simulink model "CONTROL_01"  (R2018b)
settings: Solver=FixedStepAuto  StartTime=0.0  StopTime=30  FixedStep=0.01  RelTol=1e-3
model workspace: external: MATLAB File D:\OneDrive\STUDY\RIC LAB\PROJECT 6DOF\CODE\CODE 6DOF\07_CONTROL\CONTROL_02\ROBOT_DataFile.m (data not in the file)
undefined symbols (not defined in the file or in its folder): smiData, X, Y, Z
libraries: sm_lib x35, nesl_utility x7
(part 76 of 185)

== matlab function CONTROL_01/6DOF Manipulator4/Dynamics ==
  data: t input; Fe input; dthe input; the input; Fv input; Fc input; ddthe output; m input; L input; Pic input; dt output; ex output; I input
function [ddthe,dt,ex] = DYN_6DOF(t,Fe,dthe,the,Fv,Fc,m,L,Pic,I)
e1 = the(1); e2 = the(2); e3 = the(3);
e4 = the(4); e5 = the(5); e6 = the(6);
de1 = dthe(1); de2 = dthe(2); de3 = dthe(3);
de4 = dthe(4); de5 = dthe(5); de6 = dthe(6);
x1 = Pic(1,1); y1 = Pic(1,2); z1 = Pic(1,3);
x2 = Pic(2,1); y2 = Pic(2,2); z2 = Pic(2,3);
x3 = Pic(3,1); y3 = Pic(3,2); z3 = Pic(3,3);
x4 = Pic(4,1); y4 = Pic(4,2); z4 = Pic(4,3);
x5 = Pic(5,1); y5 = Pic(5,2); z5 = Pic(5,3);
x6 = Pic(6,1); y6 = Pic(6,2); z6 = Pic(6,3);
I1xx = I(1,1); I1yy = I(1,2); I1zz = I(1,3);
I1xy = I(1,4); I1yz = I(1,5); I1zx = I(1,6);
I2xx = I(2,1); I2yy = I(2,2); I2zz = I(2,3);
I2xy = I(2,4); I2yz = I(2,5); I2zx = I(2,6);
I3xx = I(3,1); I3yy = I(3,2); I3zz = I(3,3);
I3xy = I(3,4); I3yz = I(3,5); I3zx = I(3,6);
I4xx = I(4,1); I4yy = I(4,2); I4zz = I(4,3);
I4xy = I(4,4); I4yz = I(4,5); I4zx = I(4,6);
I5xx = I(5,1); I5yy = I(5,2); I5zz = I(5,3);
I5xy = I(5,4); I5yz = I(5,5); I5zx = I(5,6);
I6xx = I(6,1); I6yy = I(6,2); I6zz = I(6,3);
I6xy = I(6,4); I6yz = I(6,5); I6zx = I(6,6);
a1 = L(1); a2 = L(2); a3 = L(3); d1 = L(4); d4 = L(5); d7 = L(6);
m1 = m(1); m2 = m(2); m3 = m(3); m4 = m(4); m5 = m(5); m6 = m(6);
g = -9.80665;
%% 
M = ...
[I1zz + m3*(cos(e1)*(a1 + a2*sin(e2)) - z3*sin(e1) + y3*cos(e2 + e3)*cos(e1) + x3*sin(e2 + e3)*cos(e1))^2 + m6*(sin(e1)*(a1 + d4*cos(e2 + e3) + a3*sin(e2 + e3) + a2*sin(e2)) - x6*(sin(e6)*(cos(e1)*cos(e4) + sin(e2 + e3)*sin(e1)*sin(e4)) + cos(e6)*(cos(e5)*(cos(e1)*sin(e4) - sin(e2 + e3)*cos(e4)*sin(e1)) - cos(e2 + e3)*sin(e1)*sin(e5))) - y6*(cos(e6)*(cos(e1)*cos(e4) + sin(e2 + e3)*sin(e1)*sin(e4)) - sin(e6)*(cos(e5)*(cos(e1)*sin(e4) - sin(e2 + e3)*cos(e4)*sin(e1)) - cos(e2 + e3)*sin(e1)*sin(e5))) + z6*(sin(e5)*(cos(e1)*sin(e4) - sin(e2 + e3)*cos(e4)*sin(e1)) + cos(e2 + e3)*cos(e5)*sin(e1)))^2 + (I6xx*(cos(e2)*cos(e3)*sin(e4)*sin(e6) + cos(e2)*cos(e6)*sin(e3)*sin(e5) + cos(e3)*cos(e6)*sin(e2)*sin(e5) - sin(e2)*sin(e3)*sin(e4)*sin(e6) - cos(e2)*cos(e3)*cos(e4)*cos(e5)*cos(e6) + cos(e4)*cos(e5)*cos(e6)*sin(e2)*sin(e3)) + I6xy*(cos(e6)*sin(e2)*sin(e3)*sin(e4) - cos(e2)*cos(e3)*cos(e6)*sin(e4) + cos(e2)*sin(e3)*sin(e5)*sin(e6) + cos(e3)*sin(e2)*sin(e5)*sin(e6) - cos(e2)*cos(e3)*cos(e4)*cos(e5)*sin(e6) + cos(e4)*cos(e5)*sin(e2)*sin(e3)*sin(e6)) - I6zx*(cos(e2)*cos(e5)*sin(e3) + cos(e3)*cos(e5)*sin(e2) + cos(e2)*cos(e3)*cos(e4)*sin(e5) - cos(e4)*sin(e2)*sin(e3)*sin(e5)))*(cos(e2)*cos(e3)*sin(e4)*sin(e6) + cos(e2)*cos(e6)*sin(e3)*sin(e5) + cos(e3)*cos(e6)*sin(e2)*sin(e5) - sin(e2)*sin(e3)*sin(e4)*sin(e6) - cos(e2)*cos(e3)*cos(e4)*cos(e5)*cos(e6) + cos(e4)*cos(e5)*cos(e6)*sin(e2)*sin(e3)) + (cos(e2)*cos(e3)*sin(e4) - sin(e2)*sin(e3)*sin(e4))*(I5zz*(cos(e2)*cos(e3)*sin(e4) - sin(e2)*sin(e3)*sin(e4)) + I5yz*(cos(e2)*cos(e5)*sin(e3) + cos(e3)*cos(e5)*sin(e2) + cos(e2)*cos(e3)*cos(e4)*sin(e5) - cos(e4)*sin(e2)*sin(e3)*sin(e5)) + I5zx*(cos(e2)*sin(e3)*sin(e5) + cos(e3)*sin(e2)*sin(e5) - cos(e2)*cos(e3)*cos(e4)*cos(e5) + cos(e4)*cos(e5)*sin(e2)*sin(e3))) + (cos(e2)*cos(e3)*cos(e4) - cos(e4)*sin(e2)*sin(e3))*(I4zx*sin(e2 + e3) + I4xx*(cos(e2)*cos(e3)*cos(e4) - cos(e4)*sin(e2)*sin(e3)) + I4xy*(cos(e2)*cos(e3)*sin(e4) - sin(e2)*sin(e3)*sin(e4))) + m3*(sin(e1)*(a1 + a2*sin(e2)) + z3*cos(e1) + y3*cos(e2 + e3)*sin(e1) + x3*sin(e2 + e3)*sin(e1))^2 + (I6xy*(cos(e2)*cos(e3)*sin(e4)*sin(e6) + cos(e2)*cos(e6)*sin(e3)*sin(e5) + cos(e3)*cos(e6)*sin(e2)*sin(e5) - sin(e2)*sin(e3)*sin(e4)*sin(e6) - cos(e2)*cos(e3)*cos(e4)*cos(e5)*cos(e6) + cos(e4)*cos(e5)*cos(e6)*sin(e2)*sin(e3)) + I6yy*(cos(e6)*sin(e2)*sin(e3)*sin(e4) - cos(e2)*cos(e3)*cos(e6)*sin(e4) + cos(e2)*sin(e3)*sin(e5)*sin(e6) + cos(e3)*sin(e2)*sin(e5)*sin(e6) - cos(e2)*cos(e3)*cos(e4)*cos(e5)*sin(e6) + cos(e4)*cos(e5)*sin(e2)*sin(e3)*sin(e6)) + I6yz*(cos(e2)*cos(e5)*sin(e3) + cos(e3)*cos(e5)*sin(e2) + cos(e2)*cos(e3)*cos(e4)*sin(e5) - cos(e4)*sin(e2)*sin(e3)*sin(e5)))*(cos(e6)*sin(e2)*sin(e3)*sin(e4) - cos(e2)*cos(e3)*cos(e6)*sin(e4) + cos(e2)*sin(e3)*sin(e5)*sin(e6) + cos(e3)*sin(e2)*sin(e5)*sin(e6) - cos(e2)*cos(e3)*cos(e4)*cos(e5)*sin(e6) + cos(e4)*cos(e5)*sin(e2)*sin(e3)*sin(e6)) + (I5zx*(cos(e2)*cos(e3)*sin(e4) - sin(e2)*sin(e3)*sin(e4)) + I5xx*(cos(e2)*sin(e3)*sin(e5) + cos(e3)*sin(e2)*sin(e5) - cos(e2)*cos(e3)*cos(e4)*cos(e5) + cos(e4)*cos(e5)*sin(e2)*sin(e3)) - I5xy*(cos(e2)*cos(e5)*sin(e3) + cos(e3)*cos(e5)*sin(e2) + cos(e2)*cos(e3)*cos(e4)*sin(e5) - cos(e4)*sin(e2)*sin(e3)*sin(e5)))*(cos(e2)*sin(e3)*sin(e5) + cos(e3)*sin(e2)*sin(e5) - cos(e2)*cos(e3)*cos(e4)*cos(e5) + cos(e4)*cos(e5)*sin(e2)*sin(e3)) + (I5yz*(cos(e2)*cos(e3)*sin(e4) - sin(e2)*sin(e3)*sin(e4)) - I5xy*(cos(e2)*sin(e3)*sin(e5) + cos(e3)*sin(e2)*sin(e5) - cos(e2)*cos(e3)*cos(e4)*cos(e5) + cos(e4)*cos(e5)*sin(e2)*sin(e3)) + I5yy*(cos(e2)*cos(e5)*sin(e3) + cos(e3)*cos(e5)*sin(e2) + cos(e2)*cos(e3)*cos(e4)*sin(e5) - cos(e4)*sin(e2)*sin(e3)*sin(e5)))*(cos(e2)*cos(e5)*sin(e3) + cos(e3)*cos(e5)*sin(e2) + cos(e2)*cos(e3)*cos(e4)*sin(e5) - cos(e4)*sin(e2)*sin(e3)*sin(e5)) + m5*(cos(e1)*(a1 + d4*cos(e2 + e3) + a3*sin(e2 + e3) + a2*sin(e2)) - z5*(cos(e4)*sin(e1) - sin(e2 + e3)*cos(e1)*sin(e4)) + x5*(cos(e5)*(sin(e1)*sin(e4) + sin(e2 + e3)*cos(e1)*cos(e4)) + cos(e2 + e3)*cos(e1)*sin(e5)) - y5*(sin(e5)*(sin(e1)*sin(e4) + sin(e2 + e3)*cos(e1)*cos(e4)) - cos(e2 + e3)*cos(e1)*cos(e5)))^2 + (cos(e2)*cos(e3)*sin(e4) - sin(e2)*sin(e3)*sin(e4))*(I4xy*(cos(e2)*cos(e3)*cos(e4) - cos(e4)*sin(e2)*sin(e3)) - I4yz*sin(e2 + e3) + I4yy*(cos(e2)*cos(e3)*sin(e4) - sin(e2)*sin(e3)*sin(e4))) + cos(e2)*(I2xx*cos(e2) + I2xy*sin(e2)) + sin(e2)*(I2xy*cos(e2) + I2yy*sin(e2)) + m4*(cos(e1)*(a1 + d4*cos(e2 + e3) + a3*sin(e2 + e3) + a2*sin(e2)) + x4*(sin(e1)*sin(e4) + sin(e2 + e3)*cos(e1)*cos(e4)) + y4*(cos(e4)*sin(e1) - sin(e2 + e3)*cos(e1)*sin(e4)) + z4*cos(e2 + e3)*cos(e1))^2 + m5*(sin(e1)*(a1 + d4*cos(e2 + e3) + a3*sin(e2 + e3) + a2*sin(e2)) + z5*(cos(e1)*cos(e4) + sin(e2 + e3)*sin(e1)*sin(e4)) - x5*(cos(e5)*(cos(e1)*sin(e4) - sin(e2 + e3)*cos(e4)*sin(e1)) - cos(e2 + e3)*sin(e1)*sin(e5)) + y5*(sin(e5)*(cos(e1)*sin(e4) - sin(e2 + e3)*cos(e4)*sin(e1)) + cos(e2 + e3)*cos(e5)*sin(e1)))^2 + m2*(a1*cos(e1) - z2*sin(e1) + y2*cos(e1)*cos(e2) + x2*cos(e1)*sin(e2))^2 + (I6yz*(cos(e6)*sin(e2)*sin(e3)*sin(e4) - cos(e2)*cos(e3)*cos(e6)*sin(e4) + cos(e2)*sin(e3)*sin(e5)*sin(e6) + cos(e3)*sin(e2)*sin(e5)*sin(e6) - cos(e2)*cos(e3)*cos(e4)*cos(e5)*sin(e6) + cos(e4)*cos(e5)*sin(e2)*sin(e3)*sin(e6)) - I6zx*(cos(e2)*cos(e3)*sin(e4)*sin(e6) + cos(e2)*cos(e6)*sin(e3)*sin(e5) + cos(e3)*cos(e6)*sin(e2)*sin(e5) - sin(e2)*sin(e3)*sin(e4)*sin(e6) - cos(e2)*cos(e3)*cos(e4)*cos(e5)*cos(e6) + cos(e4)*cos(e5)*cos(e6)*sin(e2)*sin(e3)) + I6zz*(cos(e2)*cos(e5)*sin(e3) + cos(e3)*cos(e5)*sin(e2) + cos(e2)*cos(e3)*cos(e4)*sin(e5) - cos(e4)*sin(e2)*sin(e3)*sin(e5)))*(cos(e2)*cos(e5)*sin(e3) + cos(e3)*cos(e5)*sin(e2) + cos(e2)*cos(e3)*cos(e4)*sin(e5) - cos(e4)*sin(e2)*sin(e3)*sin(e5)) + m4*(sin(e1)*(a1 + d4*cos(e2 + e3) + a3*sin(e2 + e3) + a2*sin(e2)) - x4*(cos(e1)*sin(e4) - sin(e2 + e3)*cos(e4)*sin(e1)) - y4*(cos(e1)*cos(e4) + sin(e2 + e3)*sin(e1)*sin(e4)) + z4*cos(e2 + e3)*sin(e1))^2 + cos(e2 + e3)*(I3xx*cos(e2 + e3) + I3xy*sin(e2 + e3)) + m2*(a1*sin(e1) + z2*cos(e1) + y2*cos(e2)*sin(e1) + x2*sin(e1)*sin(e2))^2 + sin(e2 + e3)*(I3xy*cos(e2 + e3) + I3yy*sin(e2 + e3)) + m1*(y1*cos(e1) + x1*sin(e1))^2 + m1*(x1*cos(e1) - y1*sin(e1))^2 + m6*(cos(e1)*(a1 + d4*cos(e2 + e3) + a3*sin(e2 + e3) + a2*sin(e2)) + x6*(sin(e6)*(cos(e4)*sin(e1) - sin(e2 + e3)*cos(e1)*sin(e4)) + cos(e6)*(cos(e5)*(sin(e1)*sin(e4) + sin(e2 + e3)*cos(e1)*cos(e4)) + cos(e2 + e3)*cos(e1)*sin(e5))) + y6*(cos(e6)*(cos(e4)*sin(e1) - sin(e2 + e3)*cos(e1)*sin(e4)) - sin(e6)*(cos(e5)*(sin(e1)*sin(e4) + sin(e2 + e3)*cos(e1)*cos(e4)) + cos(e2 + e3)*cos(e1)*sin(e5))) - z6*(sin(e5)*(sin(e1)*sin(e4) + sin(e2 + e3)*cos(e1)*cos(e4)) - cos(e2 + e3)*cos(e1)*cos(e5)))^2 + sin(e2 + e3)*(I4zz*sin(e2 + e3) + I4zx*(cos(e2)*cos(e3)*cos(e4) - cos(e4)*sin(e2)*sin(e3)) - I4yz*(cos(e2)*cos(e3)*sin(e4) - sin(e2)*sin(e3)*sin(e4))),cos(e4)*(I4xy*(cos(e2)*cos(e3)*cos(e4) - cos(e4)*sin(e2)*sin(e3)) - I4yz*sin(e2 + e3) + I4yy*(cos(e2)*cos(e3)*sin(e4) - sin(e2)*sin(e3)*sin(e4))) - sin(e4)*(I4zx*sin(e2 + e3) + I4xx*(cos(e2)*cos(e3)*cos(e4) - cos(e4)*sin(e2)*sin(e3)) + I4xy*(cos(e2)*cos(e3)*sin(e4) - sin(e2)*sin(e3)*sin(e4))) - I3zx*cos(e2 + e3) + I3yz*sin(e2 + e3) - I2zx*cos(e2) + I2yz*sin(e2) + (cos(e4)*sin(e6) + cos(e5)*cos(e6)*sin(e4))*(I6xx*(cos(e2)*cos(e3)*sin(e4)*sin(e6) + cos(e2)*cos(e6)*sin(e3)*sin(e5) + cos(e3)*cos(e6)*sin(e2)*sin(e5) - sin(e2)*sin(e3)*sin(e4)*sin(e6) - cos(e2)*cos(e3)*cos(e4)*cos(e5)*cos(e6) + cos(e4)*cos(e5)*cos(e6)*sin(e2)*sin(e3)) + I6xy*(cos(e6)*sin(e2)*sin(e3)*sin(e4) - cos(e2)*cos(e3)*cos(e6)*sin(e4) + cos(e2)*sin(e3)*sin(e5)*sin(e6) + cos(e3)*sin(e2)*sin(e5)*sin(e6) - cos(e2)*cos(e3)*cos(e4)*cos(e5)*sin(e6) + cos(e4)*cos(e5)*sin(e2)*sin(e3)*sin(e6)) - I6zx*(cos(e2)*cos(e5)*sin(e3) + cos(e3)*cos(e5)*sin(e2) + cos(e2)*cos(e3)*cos(e4)*sin(e5) - cos(e4)*sin(e2)*sin(e3)*sin(e5))) - (cos(e4)*cos(e6) - cos(e5)*sin(e4)*sin(e6))*(I6xy*(cos(e2)*cos(e3)*sin(e4)*sin(e6) + cos(e2)*cos(e6)*sin(e3)*sin(e5) + cos(e3)*cos(e6)*sin(e2)*sin(e5) - sin(e2)*sin(e3)*sin(e4)*sin(e6) - cos(e2)*cos(e3)*cos(e4)*cos(e5)*cos(e6) + cos(e4)*cos(e5)*cos(e6)*sin(e2)*sin(e3)) + I6yy*(cos(e6)*sin(e2)*sin(e3)*sin(e4) - cos(e2)*cos(e3)*cos(e6)*sin(e4) + cos(e2)*sin(e3)*sin(e5)*sin(e6) + cos(e3)*sin(e2)*sin(e5)*sin(e6) - cos(e2)*cos(e3)*cos(e4)*cos(e5)*sin(e6) + cos(e4)*cos(e5)*sin(e2)*sin(e3)*sin(e6)) + I6yz*(cos(e2)*cos(e5)*sin(e3) + cos(e3)*cos(e5)*sin(e2) + cos(e2)*cos(e3)*cos(e4)*sin(e5) - cos(e4)*sin(e2)*sin(e3)*sin(e5))) + cos(e4)*(I5zz*(cos(e2)*cos(e3)*sin(e4) - sin(e2)*sin(e3)*sin(e4)) + I5yz*(cos(e2)*cos(e5)*sin(e3) + cos(e3)*cos(e5)*sin(e2) + cos(e2)*cos(e3)*cos(e4)*sin(e5) - cos(e4)*sin(e2)*sin(e3)*sin(e5)) + I5zx*(cos(e2)*sin(e3)*sin(e5) + cos(e3)*sin(e2)*sin(e5) - cos(e2)*cos(e3)*cos(e4)*cos(e5) + cos(e4)*cos(e5)*sin(e2)*sin(e3))) - m3*(x3*cos(e2 + e3)*cos(e1) - y3*sin(e2 + e3)*cos(e1) + a2*cos(e1)*cos(e2))*(sin(e1)*(a1 + a2*sin(e2)) + z3*cos(e1) + y3*cos(e2 + e3)*sin(e1) + x3*sin(e2 + e3)*sin(e1)) + m3*(x3*cos(e2 + e3)*sin(e1) - y3*sin(e2 + e3)*sin(e1) + a2*cos(e2)*sin(e1))*(cos(e1)*(a1 + a2*sin(e2)) - z3*sin(e1) + y3*cos(e2 + e3)*cos(e1) + x3*sin(e2 + e3)*cos(e1)) + m6*(sin(e1)*(a1 + d4*cos(e2 + e3) + a3*sin(e2 + e3) + a2*sin(e2)) - x6*(sin(e6)*(cos(e1)*cos(e4) + sin(e2 + e3)*sin(e1)*sin(e4)) + cos(e6)*(cos(e5)*(cos(e1)*sin(e4) - sin(e2 + e3)*cos(e4)*sin(e1)) - cos(e2 + e3)*sin(e1)*sin(e5))) - y6*(cos(e6)*(cos(e1)*cos(e4) + sin(e2 + e3)*sin(e1)*sin(e4)) - sin(e6)*(cos(e5)*(cos(e1)*sin(e4) - sin(e2 + e3)*cos(e4)*sin(e1)) - cos(e2 + e3)*sin(e1)*sin(e5))) + z6*(sin(e5)*(cos(e1)*sin(e4) - sin(e2 + e3)*cos(e4)*sin(e1)) + cos(e2 + e3)*cos(e5)*sin(e1)))*(x6*(cos(e6)*(sin(e2 + e3)*cos(e1)*sin(e5) - cos(e2 + e3)*cos(e1)*cos(e4)*cos(e5)) + cos(e2 + e3)*cos(e1)*sin(e4)*sin(e6)) - y6*(sin(e6)*(sin(e2 + e3)*cos(e1)*sin(e5) - cos(e2 + e3)*cos(e1)*cos(e4)*cos(e5)) - cos(e2 + e3)*cos(e1)*cos(e6)*sin(e4)) + z6*(sin(e2 + e3)*cos(e1)*cos(e5) + cos(e2 + e3)*cos(e1)*cos(e4)*sin(e5)) - cos(e1)*(a3*cos(e2 + e3) - d4*sin(e2 + e3) + a2*cos(e2))) - sin(e4)*sin(e5)*(I6yz*(cos(e6)*sin(e2)*sin(e3)*sin(e4) - cos(e2)*cos(e3)*cos(e6)*sin(e4) + cos(e2)*sin(e3)*sin(e5)*sin(e6) + cos(e3)*sin(e2)*sin(e5)*sin(e6) - cos(e2)*cos(e3)*cos(e4)*cos(e5)*sin(e6) + cos(e4)*cos(e5)*sin(e2)*sin(e3)*sin(e6)) - I6zx*(cos(e2)*cos(e3)*sin(e4)*sin(e6) + cos(e2)*cos(e6)*sin(e3)*sin(e5) + cos(e3)*cos(e6)*sin(e2)*sin(e5) - sin(e2)*sin(e3)*sin(e4)*sin(e6) - cos(e2)*cos(e3)*cos(e4)*cos(e5)*cos(e6) + cos(e4)*cos(e5)*cos(e6)*sin(e2)*sin(e3)) + I6zz*(cos(e2)*cos(e5)*sin(e3) + cos(e3)*cos(e5)*sin(e2) + cos(e2)*cos(e3)*cos(e4)*sin(e5) - cos(e4)*sin(e2)*sin(e3)*sin(e5))) - m6*(cos(e1)*(a1 + d4*cos(e2 + e3) + a3*sin(e2 + e3) + a2*sin(e2)) + x6*(sin(e6)*(cos(e4)*sin(e1) - sin(e2 + e3)*cos(e1)*sin(e4)) + cos(e6)*(cos(e5)*(sin(e1)*sin(e4) + sin(e2 + e3)*cos(e1)*cos(e4)) + cos(e2 + e3)*cos(e1)*sin(e5))) + y6*(cos(e6)*(cos(e4)*sin(e1) - sin(e2 + e3)*cos(e1)*sin(e4)) - sin(e6)*(cos(e5)*(sin(e1)*sin(e4) + sin(e2 + e3)*cos(e1)*cos(e4)) + cos(e2 + e3)*cos(e1)*sin(e5))) - z6*(sin(e5)*(sin(e1)*sin(e4) + sin(e2 + e3)*cos(e1)*cos(e4)) - cos(e2 + e3)*cos(e1)*cos(e5)))*(x6*(cos(e6)*(sin(e2 + e3)*sin(e1)*sin(e5) - cos(e2 + e3)*cos(e4)*cos(e5)*sin(e1)) + cos(e2 + e3)*sin(e1)*sin(e4)*sin(e6)) - y6*(sin(e6)*(sin(e2 + e3)*sin(e1)*sin(e5) - cos(e2 + e3)*cos(e4)*cos(e5)*sin(e1)) - cos(e2 + e3)*cos(e6)*sin(e1)*sin(e4)) + z6*(sin(e2 + e3)*cos(e5)*sin(e1) + cos(e2 + e3)*cos(e4)*sin(e1)*sin(e5)) - sin(e1)*(a3*cos(e2 + e3) - d4*sin(e2 + e3) + a2*cos(e2))) + m5*(x5*(sin(e2 + e3)*cos(e1)*sin(e5) - cos(e2 + e3)*cos(e1)*cos(e4)*cos(e5)) + y5*(sin(e2 + e3)*cos(e1)*cos(e5) + cos(e2 + e3)*cos(e1)*cos(e4)*sin(e5)) - cos(e1)*(a3*cos(e2 + e3) - d4*sin(e2 + e3) + a2*cos(e2)) - z5*cos(e2 + e3)*cos(e1)*sin(e4))*(sin(e1)*(a1 + d4*cos(e2 + e3) + a3*sin(e2 + e3) + a2*sin(e2)) + z5*(cos(e1)*cos(e4) + sin(e2 + e3)*sin(e1)*sin(e4)) - x5*(cos(e5)*(cos(e1)*sin(e4) - sin(e2 + e3)*cos(e4)*sin(e1)) - cos(e2 + e3)*sin(e1)*sin(e5)) + y5*(sin(e5)*(cos(e1)*sin(e4) - sin(e2 + e3)*cos(e4)*sin(e1)) + cos(e2 + e3)*cos(e5)*sin(e1))) - m2*(x2*cos(e1)*cos(e2) - y2*cos(e1)*sin(e2))*(a1*sin(e1) + z2*cos(e1) + y2*cos(e2)*sin(e1) + x2*sin(e1)*sin(e2)) + m2*(x2*cos(e2)*sin(e1) - y2*sin(e1)*sin(e2))*(a1*cos(e1) - z2*sin(e1) + y2*cos(e1)*cos(e2) + x2*cos(e1)*sin(e2)) - m4*(cos(e1)*(a3*cos(e2 + e3) - d4*sin(e2 + e3) + a2*cos(e2)) - z4*sin(e2 + e3)*cos(e1) - y4*cos(e2 + e3)*cos(e1)*sin(e4) + x4*cos(e2 + e3)*cos(e1)*cos(e4))*(sin(e1)*(a1 + d4*cos(e2 + e3) + a3*sin(e2 + e3) + a2*sin(e2)) - x4*(cos(e1)*sin(e4) - sin(e2 + e3)*cos(e4)*sin(e1)) - y4*(cos(e1)*cos(e4) + sin(e2 + e3)*sin(e1)*sin(e4)) + z4*cos(e2 + e3)*sin(e1)) - m5*(cos(e1)*(a1 + d4*cos(e2 + e3) + a3*sin(e2 + e3) + a2*sin(e2)) - z5*(cos(e4)*sin(e1) - sin(e2 + e3)*cos(e1)*sin(e4)) + x5*(cos(e5)*(sin(e1)*sin(e4) + sin(e2 + e3)*cos(e1)*cos(e4)) + cos(e2 + e3)*cos(e1)*sin(e5)) - y5*(sin(e5)*(sin(e1)*sin(e4) + sin(e2 + e3)*cos(e1)*cos(e4)) - cos(e2 + e3)*cos(e1)*cos(e5)))*(x5*(sin(e2 + e3)*sin(e1)*sin(e5) - cos(e2 + e3)*cos(e4)*cos(e5)*sin(e1)) + y5*(sin(e2 + e3)*cos(e5)*sin(e1) + cos(e2 + e3)*cos(e4)*sin(e1)*sin(e5)) - sin(e1)*(a3*cos(e2 + e3) - d4*sin(e2 + e3) + a2*cos(e2)) - z5*cos(e2 + e3)*sin(e1)*sin(e4)) + m4*(cos(e1)*(a1 + d4*cos(e2 + e3) + a3*sin(e2 + e3) + a2*sin(e2)) + x4*(sin(e1)*sin(e4) + sin(e2 + e3)*cos(e1)*cos(e4)) + y4*(cos(e4)*sin(e1) - sin(e2 + e3)*cos(e1)*sin(e4)) + z4*cos(e2 + e3)*cos(e1))*(sin(e1)*(a3*cos(e2 + e3) - d4*sin(e2 + e3) + a2*cos(e2)) - z4*sin(e2 + e3)*sin(e1) + x4*cos(e2 + e3)*cos(e4)*sin(e1) - y4*cos(e2 + e3)*sin(e1)*sin(e4)) + cos(e5)*sin(e4)*(I5zx*(cos(e2)*cos(e3)*sin(e4) - sin(e2)*sin(e3)*sin(e4)) + I5xx*(cos(e2)*sin(e3)*sin(e5) + cos(e3)*sin(e2)*sin(e5) - cos(e2)*cos(e3)*cos(e4)*cos(e5) + cos(e4)*cos(e5)*sin(e2)*sin(e3)) - I5xy*(cos(e2)*cos(e5)*sin(e3) + cos(e3)*cos(e5)*sin(e2) + cos(e2)*cos(e3)*cos(e4)*sin(e5) - cos(e4)*sin(e2)*sin(e3)*sin(e5))) - sin(e4)*sin(e5)*(I5yz*(cos(e2)*cos(e3)*sin(e4) - sin(e2)*sin(e3)*sin(e4)) - I5xy*(cos(e2)*sin(e3)*sin(e5) + cos(e3)*sin(e2)*sin(e5) - cos(e2)*cos(e3)*cos(e4)*cos(e5) + cos(e4)*cos(e5)*sin(e2)*sin(e3)) + I5yy*(cos(e2)*cos(e5)*sin(e3) + cos(e3)*cos(e5)*sin(e2) + cos(e2)*cos(e3)*cos(e4)*sin(e5) - cos(e4)*sin(e2)*sin(e3)*sin(e5))),cos(e4)*(I4xy*(cos(e2)*cos(e3)*cos(e4) - cos(e4)*sin(e2)*sin(e3)) - I4yz*sin(e2 + e3) + I4yy*(cos(e2)*cos(e3)*sin(e4) - sin(e2)*sin(e3)*sin(e4))) - sin(e4)*(I4zx*sin(e2 + e3) + I4xx*(cos(e2)*cos(e3)*cos(e4) - cos(e4)*sin(e2)*sin(e3)) + I4xy*(cos(e2)*cos(e3)*sin(e4) - sin(e2)*sin(e3)*sin(e4))) - I3zx*cos(e2 + e3) + I3yz*sin(e2 + e3) + (cos(e4)*sin(e6) + cos(e5)*cos(e6)*sin(e4))*(I6xx*(cos(e2)*cos(e3)*sin(e4)*sin(e6) + cos(e2)*cos(e6)*sin(e3)*sin(e5) + cos(e3)*cos(e6)*sin(e2)*sin(e5) - sin(e2)*sin(e3)*sin(e4)*sin(e6) - cos(e2)*cos(e3)*cos(e4)*cos(e5)*cos(e6) + cos(e4)*cos(e5)*cos(e6)*sin(e2)*sin(e3)) + I6xy*(cos(e6)*sin(e2)*sin(e3)*sin(e4) - cos(e2)*cos(e3)*cos(e6)*sin(e4) + cos(e2)*sin(e3)*sin(e5)*sin(e6) + cos(e3)*sin(e2)*sin(e5)*sin(e6) - cos(e2)*cos(e3)*cos(e4)*cos(e5)*sin(e6) + cos(e4)*cos(e5)*sin(e2)*sin(e3)*sin(e6)) - I6zx*(cos(e2)*cos(e5)*sin(e3) + cos(e3)*cos(e5)*sin(e2) + cos(e2)*cos(e3)*cos(e4)*sin(e5) - cos(e4)*sin(e2)*sin(e3)*sin(e5))) - (cos(e4)*cos(e6) - cos(e5)*sin(e4)*sin(e6))*(I6xy*(cos(e2)*cos(e3)*sin(e4)*sin(e6) + cos(e2)*cos(e6)*sin(e3)*sin(e5) + cos(e3)*cos(e6)*sin(e2)*sin(e5) - sin(e2)*sin(e3)*sin(e4)*sin(e6) - cos(e2)*cos(e3)*cos(e4)*cos(e5)*cos(e6) + cos(e4)*cos(e5)*cos(e6)*sin(e2)*sin(e3)) + I6yy*(cos(e6)*sin(e2)*sin(e3)*sin(e4) - cos(e2)*cos(e3)*cos(e6)*sin(e4) + cos(e2)*sin(e3)*sin(e5)*sin(e6) + cos(e3)*sin(e2)*sin(e5)*sin(e6) - cos(e2)*cos(e3)*cos(e4)*cos(e5)*sin(e6) + cos(e4)*cos(e5)*sin(e2)*sin(e3)*sin(e6)) + I6yz*(cos(e2)*cos(e5)*sin(e3) + cos(e3)*cos(e5)*sin(e2) + cos(e2)*cos(e3)*cos(e4)*sin(e5) - cos(e4)*sin(e2)*sin(e3)*sin(e5))) + cos(e4)*(I5zz*(cos(e2)*cos(e3)*sin(e4) - sin(e2)*sin(e3)*sin(e4)) + I5yz*(cos(e2)*cos(e5)*sin(e3) + cos(e3)*cos(e5)*sin(e2) + cos(e2)*cos(e3)*cos(e4)*sin(e5) - cos(e4)*sin(e2)*sin(e3)*sin(e5)) + I5zx*(cos(e2)*sin(e3)*sin(e5) + cos(e3)*sin(e2)*sin(e5) - cos(e2)*cos(e3)*cos(e4)*cos(e5) + cos(e4)*cos(e5)*sin(e2)*sin(e3))) + m5*(sin(e1)*(a1 + d4*cos(e2 + e3) + a3*sin(e2 + e3) + a2*sin(e2)) + z5*(cos(e1)*cos(e4) + sin(e2 + e3)*sin(e1)*sin(e4)) - x5*(cos(e5)*(cos(e1)*sin(e4) - sin(e2 + e3)*cos(e4)*sin(e1)) - cos(e2 + e3)*sin(e1)*sin(e5)) + y5*(sin(e5)*(cos(e1)*sin(e4) - sin(e2 + e3)*cos(e4)*sin(e1)) + cos(e2 + e3)*cos(e5)*sin(e1)))*(x5*(sin(e2 + e3)*cos(e1)*sin(e5) - cos(e2 + e3)*cos(e1)*cos(e4)*cos(e5)) + y5*(sin(e2 + e3)*cos(e1)*cos(e5) + cos(e2 + e3)*cos(e1)*cos(e4)*sin(e5)) - cos(e1)*(a3*cos(e2 + e3) - d4*sin(e2 + e3)) - z5*cos(e2 + e3)*cos(e1)*sin(e4)) - m4*(sin(e1)*(a1 + d4*cos(e2 + e3) + a3*sin(e2 + e3) + a2*sin(e2)) - x4*(cos(e1)*sin(e4) - sin(e2 + e3)*cos(e4)*sin(e1)) - y4*(cos(e1)*cos(e4) + sin(e2 + e3)*sin(e1)*sin(e4)) + z4*cos(e2 + e3)*sin(e1))*(cos(e1)*(a3*cos(e2 + e3) - d4*sin(e2 + e3)) - z4*sin(e2 + e3)*cos(e1) - y4*cos(e2 + e3)*cos(e1)*sin(e4) + x4*cos(e2 + e3)*cos(e1)*cos(e4)) - sin(e4)*sin(e5)*(I6yz*(cos(e6)*sin(e2)*sin(e3)*sin(e4) - cos(e2)*cos(e3)*cos(e6)*sin(e4) + cos(e2)*sin(e3)*sin(e5)*sin(e6) + cos(e3)*sin(e2)*sin(e5)*sin(e6) - cos(e2)*cos(e3)*cos(e4)*cos(e5)*sin(e6) + cos(e4)*cos(e5)*sin(e2)*sin(e3)*sin(e6)) - I6zx*(cos(e2)*cos(e3)*sin(e4)*sin(e6) + cos(e2)*cos(e6)*sin(e3)*sin(e5) + cos(e3)*cos(e6)*sin(e2)*sin(e5) - sin(e2)*sin(e3)*sin(e4)*sin(e6) - cos(e2)*cos(e3)*cos(e4)*cos(e5)*cos(e6) + cos(e4)*cos(e5)*cos(e6)*sin(e2)*sin(e3)) + I6zz*(cos(e2)*cos(e5)*sin(e3) + cos(e3)*cos(e5)*sin(e2) + cos(e2)*cos(e3)*cos(e4)*sin(e5) - cos(e4)*sin(e2)*sin(e3)*sin(e5))) - m5*(x5*(sin(e2 + e3)*sin(e1)*sin(e5) - cos(e2 + e3)*cos(e4)*cos(e5)*sin(e1)) + y5*(sin(e2 + e3)*cos(e5)*sin(e1) + cos(e2 + e3)*cos(e4)*sin(e1)*sin(e5)) - sin(e1)*(a3*cos(e2 + e3) - d4*sin(e2 + e3)) - z5*cos(e2 + e3)*sin(e1)*sin(e4))*(cos(e1)*(a1 + d4*cos(e2 + e3) + a3*sin(e2 + e3) + a2*sin(e2)) - z5*(cos(e4)*sin(e1) - sin(e2 + e3)*cos(e1)*sin(e4)) + x5*(cos(e5)*(sin(e1)*sin(e4) + sin(e2 + e3)*cos(e1)*cos(e4)) + cos(e2 + e3)*cos(e1)*sin(e5)) - y5*(sin(e5)*(sin(e1)*sin(e4) + sin(e2 + e3)*cos(e1)*cos(e4)) - cos(e2 + e3)*cos(e1)*cos(e5))) + m4*(sin(e1)*(a3*cos(e2 + e3) - d4*sin(e2 + e3)) - z4*sin(e2 + e3)*sin(e1) + x4*cos(e2 + e3)*cos(e4)*sin(e1) - y4*cos(e2 + e3)*sin(e1)*sin(e4))*(cos(e1)*(a1 + d4*cos(e2 + e3) + a3*sin(e2 + e3) + a2*sin(e2)) + x4*(sin(e1)*sin(e4) + sin(e2 + e3)*cos(e1)*cos(e4)) + y4*(cos(e4)*sin(e1) - sin(e2 + e3)*cos(e1)*sin(e4)) + z4*cos(e2 + e3)*cos(e1)) + m6*(sin(e1)*(a1 + d4*cos(e2 + e3) + a3*sin(e2 + e3) + a2*sin(e2)) - x6*(sin(e6)*(cos(e1)*cos(e4) + sin(e2 + e3)*sin(e1)*sin(e4)) + cos(e6)*(cos(e5)*(cos(e1)*sin(e4) - sin(e2 + e3)*cos(e4)*sin(e1)) - cos(e2 + e3)*sin(e1)*sin(e5))) - y6*(cos(e6)*(cos(e1)*cos(e4) + sin(e2 + e3)*sin(e1)*sin(e4)) - sin(e6)*(cos(e5)*(cos(e1)*sin(e4) - sin(e2 + e3)*cos(e4)*sin(e1)) - cos(e2 + e3)*sin(e1)*sin(e5))) + z6*(sin(e5)*(cos(e1)*sin(e4) - sin(e2 + e3)*cos(e4)*sin(e1)) + cos(e2 + e3)*cos(e5)*sin(e1)))*(x6*(cos(e6)*(sin(e2 + e3)*cos(e1)*sin(e5) - cos(e2 + e3)*cos(e1)*cos(e4)*cos(e5)) + cos(e2 + e3)*cos(e1)*sin(e4)*sin(e6)) - y6*(sin(e6)*(sin(e2 + e3)*cos(e1)*sin(e5) - cos(e2 + e3)*cos(e1)*cos(e4)*cos(e5)) - cos(e2 + e3)*cos(e1)*cos(e6)*sin(e4)) + z6*(sin(e2 + e3)*cos(e1)*cos(e5) + cos(e2 + e3)*cos(e1)*cos(e4)*sin(e5)) - cos(e1)*(a3*cos(e2 + e3) - d4*sin(e2 + e3))) - m3*(x3*cos(e2 + e3)*cos(e1) - y3*sin(e2 + e3)*cos(e1))*(sin(e1)*(a1 + a2*sin(e2)) + z3*cos(e1) + y3*cos(e2 + e3)*sin(e1) + x3*sin(e2 + e3)*sin(e1)) + m3*(x3*cos(e2 + e3)*sin(e1) - y3*sin(e2 + e3)*sin(e1))*(cos(e1)*(a1 + a2*sin(e2)) - z3*sin(e1) + y3*cos(e2 + e3)*cos(e1) + x3*sin(e2 + e3)*cos(e1)) + cos(e5)*sin(e4)*(I5zx*(cos(e2)*cos(e3)*sin(e4) - sin(e2)*sin(e3)*sin(e4)) + I5xx*(cos(e2)*sin(e3)*sin(e5) + cos(e3)*sin(e2)*sin(e5) - cos(e2)*cos(e3)*cos(e4)*cos(e5) + cos(e4)*cos(e5)*sin(e2)*sin(e3)) - I5xy*(cos(e2)*cos(e5)*sin(e3) + cos(e3)*cos(e5)*sin(e2) + cos(e2)*cos(e3)*cos(e4)*sin(e5) - cos(e4)*sin(e2)*sin(e3)*sin(e5))) - m6*(x6*(cos(e6)*(sin(e2 + e3)*sin(e1)*sin(e5) - cos(e2 + e3)*cos(e4)*cos(e5)*sin(e1)) + cos(e2 + e3)*sin(e1)*sin(e4)*sin(e6)) - y6*(sin(e6)*(sin(e2 + e3)*sin(e1)*sin(e5) - cos(e2 + e3)*cos(e4)*cos(e5)*sin(e1)) - cos(e2 + e3)*cos(e6)*sin(e1)*sin(e4)) + z6*(sin(e2 + e3)*cos(e5)*sin(e1) + cos(e2 + e3)*cos(e4)*sin(e1)*sin(e5)) - sin(e1)*(a3*cos(e2 + e3) - d4*sin(e2 + e3)))*(cos(e1)*(a1 + d4*cos(e2 + e3) + a3*sin(e2 + e3) + a2*sin(e2)) + x6*(sin(e6)*(cos(e4)*sin(e1) - sin(e2 + e3)*cos(e1)*sin(e4)) + cos(e6)*(cos(e5)*(sin(e1)*sin(e4) + sin(e2 + e3)*cos(e1)*cos(e4)) + cos(e2 + e3)*cos(e1)*sin(e5))) + y6*(cos(e6)*(cos(e4)*sin(e1) - sin(e2 + e3)*cos(e1)*sin(e4)) - sin(e6)*(cos(e5)*(sin(e1)*sin(e4) + sin(e2 + e3)*cos(e1)*cos(e4)) + cos(e2 + e3)*cos(e1)*sin(e5))) - z6*(sin(e5)*(sin(e1)*sin(e4) + sin(e2 + e3)*cos(e1)*cos(e4)) - cos(e2 + e3)*cos(e1)*cos(e5))) - sin(e4)*sin(e5)*(I5yz*(cos(e2)*cos(e3)*sin(e4) - sin(e2)*sin(e3)*sin(e4)) - I5xy*(cos(e2)*sin(e3)*sin(e5) + cos(e3)*sin(e2)*sin(e5) - cos(e2)*cos(e3)*cos(e4)*cos(e5) + cos(e4)*cos(e5)*sin(e2)*sin(e3)) + I5yy*(cos(e2)*cos(e5)*sin(e3) + cos(e3)*cos(e5)*sin(e2) + cos(e2)*cos(e3)*cos(e4)*sin(e5) - cos(e4)*sin(e2)*sin(e3)*sin(e5))),I4yz*(cos(e2)*cos(e3)*sin(e4) - sin(e2)*sin(e3)*sin(e4)) - cos(e5)*(I6yz*(cos(e6)*sin(e2)*sin(e3)*sin(e4) - cos(e2)*cos(e3)*cos(e6)*sin(e4) + cos(e2)*sin(e3)*sin(e5)*sin(e6) + cos(e3)*sin(e2)*sin(e5)*sin(e6) - cos(e2)*cos(e3)*cos(e4)*cos(e5)*sin(e6) + cos(e4)*cos(e5)*sin(e2)*sin(e3)*sin(e6)) - I6zx*(cos(e2)*cos(e3)*sin(e4)*sin(e6) + cos(e2)*cos(e6)*sin(e3)*sin(e5) + cos(e3)*cos(e6)*sin(e2)*sin(e5) - sin(e2)*sin(e3)*sin(e4)*sin(e6) - cos(e2)*cos(e3)*cos(e4)*cos(e5)*cos(e6) + cos(e4)*cos(e5)*cos(e6)*sin(e2)*sin(e3)) + I6zz*(cos(e2)*cos(e5)*sin(e3) + cos(e3)*cos(e5)*sin(e2) + cos(e2)*cos(e3)*cos(e4)*sin(e5) - cos(e4)*sin(e2)*sin(e3)*sin(e5))) - I4zz*sin(e2 + e3) - I4zx*(cos(e2)*cos(e3)*cos(e4) - cos(e4)*sin(e2)*sin(e3)) - sin(e5)*(I5zx*(cos(e2)*cos(e3)*sin(e4) - sin(e2)*sin(e3)*sin(e4)) + I5xx*(cos(e2)*sin(e3)*sin(e5) + cos(e3)*sin(e2)*sin(e5) - cos(e2)*cos(e3)*cos(e4)*cos(e5) + cos(e4)*cos(e5)*sin(e2)*sin(e3)) - I5xy*(cos(e2)*cos(e5)*sin(e3) + cos(e3)*cos(e5)*sin(e2) + cos(e2)*cos(e3)*cos(e4)*sin(e5) - cos(e4)*sin(e2)*sin(e3)*sin(e5))) - cos(e5)*(I5yz*(cos(e2)*cos(e3)*sin(e4) - sin(e2)*sin(e3)*sin(e4)) - I5xy*(cos(e2)*sin(e3)*sin(e5) + cos(e3)*sin(e2)*sin(e5) - cos(e2)*cos(e3)*cos(e4)*cos(e5) + cos(e4)*cos(e5)*sin(e2)*sin(e3)) + I5yy*(cos(e2)*cos(e5)*sin(e3) + cos(e3)*cos(e5)*sin(e2) + cos(e2)*cos(e3)*cos(e4)*sin(e5) - cos(e4)*sin(e2)*sin(e3)*sin(e5))) - cos(e6)*sin(e5)*(I6xx*(cos(e2)*cos(e3)*sin(e4)*sin(e6) + cos(e2)*cos(e6)*sin(e3)*sin(e5) + cos(e3)*cos(e6)*sin(e2)*sin(e5) - sin(e2)*sin(e3)*sin(e4)*sin(e6) - cos(e2)*cos(e3)*cos(e4)*cos(e5)*cos(e6) + cos(e4)*cos(e5)*cos(e6)*sin(e2)*sin(e3)) + I6xy*(cos(e6)*sin(e2)*sin(e3)*sin(e4) - cos(e2)*cos(e3)*cos(e6)*sin(e4) + cos(e2)*sin(e3)*sin(e5)*sin(e6) + cos(e3)*sin(e2)*sin(e5)*sin(e6) - cos(e2)*cos(e3)*cos(e4)*cos(e5)*sin(e6) + cos(e4)*cos(e5)*sin(e2)*sin(e3)*sin(e6)) - I6zx*(cos(e2)*cos(e5)*sin(e3) + cos(e3)*cos(e5)*sin(e2) + cos(e2)*cos(e3)*cos(e4)*sin(e5) - cos(e4)*sin(e2)*sin(e3)*sin(e5))) - sin(e5)*sin(e6)*(I6xy*(cos(e2)*cos(e3)*sin(e4)*sin(e6) + cos(e2)*cos(e6)*sin(e3)*sin(e5) + cos(e3)*cos(e6)*sin(e2)*sin(e5) - sin(e2)*sin(e3)*sin(e4)*sin(e6) - cos(e2)*cos(e3)*cos(e4)*cos(e5)*cos(e6) + cos(e4)*cos(e5)*cos(e6)*sin(e2)*sin(e3)) + I6yy*(cos(e6)*sin(e2)*sin(e3)*sin(e4) - cos(e2)*cos(e3)*cos(e6)*sin(e4) + cos(e2)*sin(e3)*sin(e5)*sin(e6) + cos(e3)*sin(e2)*sin(e5)*sin(e6) - cos(e2)*cos(e3)*cos(e4)*cos(e5)*sin(e6) + cos(e4)*cos(e5)*sin(e2)*sin(e3)*sin(e6)) + I6yz*(cos(e2)*cos(e5)*sin(e3) + cos(e3)*cos(e5)*sin(e2) + cos(e2)*cos(e3)*cos(e4)*sin(e5) - cos(e4)*sin(e2)*sin(e3)*sin(e5))) - m4*(x4*(cos(e1)*cos(e4) + sin(e2 + e3)*sin(e1)*sin(e4)) - y4*(cos(e1)*sin(e4) - sin(e2 + e3)*cos(e4)*sin(e1)))*(cos(e1)*(a1 + d4*cos(e2 + e3) + a3*sin(e2 + e3) + a2*sin(e2)) + x4*(sin(e1)*sin(e4) + sin(e2 + e3)*cos(e1)*cos(e4)) + y4*(cos(e4)*sin(e1) - sin(e2 + e3)*cos(e1)*sin(e4)) + z4*cos(e2 + e3)*cos(e1)) + m6*(x6*(sin(e6)*(cos(e1)*sin(e4) - sin(e2 + e3)*cos(e4)*sin(e1)) - cos(e5)*cos(e6)*(cos(e1)*cos(e4) + sin(e2 + e3)*sin(e1)*sin(e4))) + y6*(cos(e6)*(cos(e1)*sin(e4) - sin(e2 + e3)*cos(e4)*sin(e1)) + cos(e5)*sin(e6)*(cos(e1)*cos(e4) + sin(e2 + e3)*sin(e1)*sin(e4))) + z6*sin(e5)*(cos(e1)*cos(e4) + sin(e2 + e3)*sin(e1)*sin(e4)))*(cos(e1)*(a1 + d4*cos(e2 + e3) + a3*sin(e2 + e3) + a2*sin(e2)) + x6*(sin(e6)*(cos(e4)*sin(e1) - sin(e2 + e3)*cos(e1)*sin(e4)) + cos(e6)*(cos(e5)*(sin(e1)*sin(e4) + sin(e2 + e3)*cos(e1)*cos(e4)) + cos(e2 + e3)*cos(e1)*sin(e5))) + y6*(cos(e6)*(cos(e4)*sin(e1) - sin(e2 + e3)*cos(e1)*sin(e4)) - sin(e6)*(cos(e5)*(sin(e1)*sin(e4) + sin(e2 + e3)*cos(e1)*cos(e4)) + cos(e2 + e3)*cos(e1)*sin(e5))) - z6*(sin(e5)*(sin(e1)*sin(e4) + sin(e2 + e3)*cos(e1)*cos(e4)) - cos(e2 + e3)*cos(e1)*cos(e5))) - m4*(x4*(cos(e4)*sin(e1) - sin(e2 + e3)*cos(e1)*sin(e4)) - y4*(sin(e1)*sin(e4) + sin(e2 + e3)*cos(e1)*cos(e4)))*(sin(e1)*(a1 + d4*cos(e2 + e3) + a3*sin(e2 + e3) + a2*sin(e2)) - x4*(cos(e1)*sin(e4) - sin(e2 + e3)*cos(e4)*sin(e1)) - y4*(cos(e1)*cos(e4) + sin(e2 + e3)*sin(e1)*sin(e4)) + z4*cos(e2 + e3)*sin(e1)) - m5*(z5*(cos(e1)*sin(e4) - sin(e2 + e3)*cos(e4)*sin(e1)) + x5*cos(e5)*(cos(e1)*cos(e4) + sin(e2 + e3)*sin(e1)*sin(e4)) - y5*sin(e5)*(cos(e1)*cos(e4) + sin(e2 + e3)*sin(e1)*sin(e4)))*(cos(e1)*(a1 + d4*cos(e2 + e3) + a3*sin(e2 + e3) + a2*sin(e2)) - z5*(cos(e4)*sin(e1) - sin(e2 + e3)*cos(e1)*sin(e4)) + x5*(cos(e5)*(sin(e1)*sin(e4) + sin(e2 + e3)*cos(e1)*cos(e4)) + cos(e2 + e3)*cos(e1)*sin(e5)) - y5*(sin(e5)*(sin(e1)*sin(e4) + sin(e2 + e3)*cos(e1)*cos(e4)) - cos(e2 + e3)*cos(e1)*cos(e5))) + m6*(x6*(sin(e6)*(sin(e1)*sin(e4) + sin(e2 + e3)*cos(e1)*cos(e4)) - cos(e5)*cos(e6)*(cos(e4)*sin(e1) - sin(e2 + e3)*cos(e1)*sin(e4))) + y6*(cos(e6)*(sin(e1)*sin(e4) + sin(e2 + e3)*cos(e1)*cos(e4)) + cos(e5)*sin(e6)*(cos(e4)*sin(e1) - sin(e2 + e3)*cos(e1)*sin(e4))) + z6*sin(e5)*(cos(e4)*sin(e1) - sin(e2 + e3)*cos(e1)*sin(e4)))*(sin(e1)*(a1 + d4*cos(e2 + e3) + a3*sin(e2 + e3) + a2*sin(e2)) - x6*(sin(e6)*(cos(e1)*cos(e4) + sin(e2 + e3)*sin(e1)*sin(e4)) + cos(e6)*(cos(e5)*(cos(e1)*sin(e4) - sin(e2 + e3)*cos(e4)*sin(e1)) - cos(e2 + e3)*sin(e1)*sin(e5))) - y6*(cos(e6)*(cos(e1)*cos(e4) + sin(e2 + e3)*sin(e1)*sin(e4)) - sin(e6)*(cos(e5)*(cos(e1)*sin(e4) - sin(e2 + e3)*cos(e4)*sin(e1)) - cos(e2 + e3)*sin(e1)*sin(e5))) + z6*(sin(e5)*(cos(e1)*sin(e4) - sin(e2 + e3)*cos(e4)*sin(e1)) + cos(e2 + e3)*cos(e5)*sin(e1))) - m5*(z5*(sin(e1)*sin(e4) + sin(e2 + e3)*cos(e1)*cos(e4)) + x5*cos(e5)*(cos(e4)*sin(e1) - sin(e2 + e3)*cos(e1)*sin(e4)) - y5*sin(e5)*(cos(e4)*sin(e1) - sin(e2 + e3)*cos(e1)*sin(e4)))*(sin(e1)*(a1 + d4*cos(e2 + e3) + a3*sin(e2 + e3) + a2*sin(e2)) + z5*(cos(e1)*cos(e4) + sin(e2 + e3)*sin(e1)*sin(e4)) - x5*(cos(e5)*(cos(e1)*sin(e4) - sin(e2 + e3)*cos(e4)*sin(e1)) - cos(e2 + e3)*sin(e1)*sin(e5)) + y5*(sin(e5)*(cos(e1)*sin(e4) - sin(e2 + e3)*cos(e4)*sin(e1)) + cos(e2 + e3)*cos(e5)*sin(e1))),sin(e6)*(I6xx*(cos(e2)*cos(e3)*sin(e4)*sin(e6) + cos(e2)*cos(e6)*sin(e3)*sin(e5) + cos(e3)*cos(e6)*sin(e2)*sin(e5) - sin(e2)*sin(e3)*sin(e4)*sin(e6) - cos(e2)*cos(e3)*cos(e4)*cos(e5)*cos(e6) + cos(e4)*cos(e5)*cos(e6)*sin(e2)*sin(e3)) + I6xy*(cos(e6)*sin(e2)*sin(e3)*sin(e4) - cos(e2)*cos(e3)*cos(e6)*sin(e4) + cos(e2)*sin(e3)*sin(e5)*sin(e6) + cos(e3)*sin(e2)*sin(e5)*sin(e6) - cos(e2)*cos(e3)*cos(e4)*cos(e5)*sin(e6) + cos(e4)*cos(e5)*sin(e2)*sin(e3)*sin(e6)) - I6zx*(cos(e2)*cos(e5)*sin(e3) + cos(e3)*cos(e5)*sin(e2) + cos(e2)*cos(e3)*cos(e4)*sin(e5) - cos(e4)*sin(e2)*sin(e3)*sin(e5))) - cos(e6)*(I6xy*(cos(e2)*cos(e3)*sin(e4)*sin(e6) + cos(e2)*cos(e6)*sin(e3)*sin(e5) + cos(e3)*cos(e6)*sin(e2)*sin(e5) - sin(e2)*sin(e3)*sin(e4)*sin(e6) - cos(e2)*cos(e3)*cos(e4)*cos(e5)*cos(e6) + cos(e4)*cos(e5)*cos(e6)*sin(e2)*sin(e3)) + I6yy*(cos(e6)*sin(e2)*sin(e3)*sin(e4) - cos(e2)*cos(e3)*cos(e6)*sin(e4) + cos(e2)*sin(e3)*sin(e5)*sin(e6) + cos(e3)*sin(e2)*sin(e5)*sin(e6) - cos(e2)*cos(e3)*cos(e4)*cos(e5)*sin(e6) + cos(e4)*cos(e5)*sin(e2)*sin(e3)*sin(e6)) + I6yz*(cos(e2)*cos(e5)*sin(e3) + cos(e3)*cos(e5)*sin(e2) + cos(e2)*cos(e3)*cos(e4)*sin(e5) - cos(e4)*sin(e2)*sin(e3)*sin(e5))) + I5zz*(cos(e2)*cos(e3)*sin(e4) - sin(e2)*sin(e3)*sin(e4)) + I5yz*(cos(e2)*cos(e5)*sin(e3) + cos(e3)*cos(e5)*sin(e2) + cos(e2)*cos(e3)*cos(e4)*sin(e5) - cos(e4)*sin(e2)*sin(e3)*sin(e5)) + I5zx*(cos(e2)*sin(e3)*sin(e5) + cos(e3)*sin(e2)*sin(e5) - cos(e2)*cos(e3)*cos(e4)*cos(e5) + cos(e4)*cos(e5)*sin(e2)*sin(e3)) + m5*(x5*(sin(e5)*(cos(e1)*sin(e4) - sin(e2 + e3)*cos(e4)*sin(e1)) + cos(e2 + e3)*cos(e5)*sin(e1)) + y5*(cos(e5)*(cos(e1)*sin(e4) - sin(e2 + e3)*cos(e4)*sin(e1)) - cos(e2 + e3)*sin(e1)*sin(e5)))*(cos(e1)*(a1 + d4*cos(e2 + e3) + a3*sin(e2 + e3) + a2*sin(e2)) - z5*(cos(e4)*sin(e1) - sin(e2 + e3)*cos(e1)*sin(e4)) + x5*(cos(e5)*(sin(e1)*sin(e4) + sin(e2 + e3)*cos(e1)*cos(e4)) + cos(e2 + e3)*cos(e1)*sin(e5)) - y5*(sin(e5)*(sin(e1)*sin(e4) + sin(e2 + e3)*cos(e1)*cos(e4)) - cos(e2 + e3)*cos(e1)*cos(e5))) + m5*(x5*(sin(e5)*(sin(e1)*sin(e4) + sin(e2 + e3)*cos(e1)*cos(e4)) - cos(e2 + e3)*cos(e1)*cos(e5)) + y5*(cos(e5)*(sin(e1)*sin(e4) + sin(e2 + e3)*cos(e1)*cos(e4)) + cos(e2 + e3)*cos(e1)*sin(e5)))*(sin(e1)*(a1 + d4*cos(e2 + e3) + a3*sin(e2 + e3) + a2*sin(e2)) + z5*(cos(e1)*cos(e4) + sin(e2 + e3)*sin(e1)*sin(e4)) - x5*(cos(e5)*(cos(e1)*sin(e4) - sin(e2 + e3)*cos(e4)*sin(e1)) - cos(e2 + e3)*sin(e1)*sin(e5)) + y5*(sin(e5)*(cos(e1)*sin(e4) - sin(e2 + e3)*cos(e4)*sin(e1)) + cos(e2 + e3)*cos(e5)*sin(e1))) + m6*(z6*(cos(e5)*(cos(e1)*sin(e4) - sin(e2 + e3)*cos(e4)*sin(e1)) - cos(e2 + e3)*sin(e1)*sin(e5)) + x6*cos(e6)*(sin(e5)*(cos(e1)*sin(e4) - sin(e2 + e3)*cos(e4)*sin(e1)) + cos(e2 + e3)*cos(e5)*sin(e1)) - y6*sin(e6)*(sin(e5)*(cos(e1)*sin(e4) - sin(e2 + e3)*cos(e4)*sin(e1)) + cos(e2 + e3)*cos(e5)*sin(e1)))*(cos(e1)*(a1 + d4*cos(e2 + e3) + a3*sin(e2 + e3) + a2*sin(e2)) + x6*(sin(e6)*(cos(e4)*sin(e1) - sin(e2 + e3)*cos(e1)*sin(e4)) + cos(e6)*(cos(e5)*(sin(e1)*sin(e4) + sin(e2 + e3)*cos(e1)*cos(e4)) + cos(e2 + e3)*cos(e1)*sin(e5))) + y6*(cos(e6)*(cos(e4)*sin(e1) - sin(e2 + e3)*cos(e1)*sin(e4)) - sin(e6)*(cos(e5)*(sin(e1)*sin(e4) + sin(e2 + e3)*cos(e1)*cos(e4)) + cos(e2 + e3)*cos(e1)*sin(e5))) - z6*(sin(e5)*(sin(e1)*sin(e4) + sin(e2 + e3)*cos(e1)*cos(e4)) - cos(e2 + e3)*cos(e1)*cos(e5))) + m6*(z6*(cos(e5)*(sin(e1)*sin(e4) + sin(e2 + e3)*cos(e1)*cos(e4)) + cos(e2 + e3)*cos(e1)*sin(e5)) + x6*cos(e6)*(sin(e5)*(sin(e1)*sin(e4) + sin(e2 + e3)*cos(e1)*cos(e4)) - cos(e2 + e3)*cos(e1)*cos(e5)) - y6*sin(e6)*(sin(e5)*(sin(e1)*sin(e4) + sin(e2 + e3)*cos(e1)*cos(e4)) - cos(e2 + e3)*cos(e1)*cos(e5)))*(sin(e1)*(a1 + d4*cos(e2 + e3) + a3*sin(e2 + e3) + a2*sin(e2)) - x6*(sin(e6)*(cos(e1)*cos(e4) + sin(e2 + e3)*sin(e1)*sin(e4)) + cos(e6)*(cos(e5)*(cos(e1)*sin(e4) - sin(e2 + e3)*cos(e4)*sin(e1)) - cos(e2 + e3)*sin(e1)*sin(e5))) - y6*(cos(e6)*(cos(e1)*cos(e4) + sin(e2 + e3)*sin(e1)*sin(e4)) - sin(e6)*(cos(e5)*(cos(e1)*sin(e4) - sin(e2 + e3)*cos(e4)*sin(e1)) - cos(e2 + e3)*sin(e1)*sin(e5))) + z6*(sin(e5)*(cos(e1)*sin(e4) - sin(e2 + e3)*cos(e4)*sin(e1)) + cos(e2 + e3)*cos(e5)*sin(e1))),I6zx*(cos(e2)*cos(e3)*sin(e4)*sin(e6) + cos(e2)*cos(e6)*sin(e3)*sin(e5) + cos(e3)*cos(e6)*sin(e2)*sin(e5) - sin(e2)*sin(e3)*sin(e4)*sin(e6) - cos(e2)*cos(e3)*cos(e4)*cos(e5)*cos(e6) + cos(e4)*cos(e5)*cos(e6)*sin(e2)*sin(e3)) - I6yz*(cos(e6)*sin(e2)*sin(e3)*sin(e4) - cos(e2)*cos(e3)*cos(e6)*sin(e4) + cos(e2)*sin(e3)*sin(e5)*sin(e6) + cos(e3)*sin(e2)*sin(e5)*sin(e6) - cos(e2)*cos(e3)*cos(e4)*cos(e5)*sin(e6) + cos(e4)*cos(e5)*sin(e2)*sin(e3)*sin(e6)) - I6zz*(cos(e2)*cos(e5)*sin(e3) + cos(e3)*cos(e5)*sin(e2) + cos(e2)*cos(e3)*cos(e4)*sin(e5) - cos(e4)*sin(e2)*sin(e3)*sin(e5)) - m6*(x6*(cos(e6)*(cos(e1)*cos(e4) + sin(e2 + e3)*sin(e1)*sin(e4)) - sin(e6)*(cos(e5)*(cos(e1)*sin(e4) - sin(e2 + e3)*cos(e4)*sin(e1)) - cos(e2 + e3)*sin(e1)*sin(e5))) - y6*(sin(e6)*(cos(e1)*cos(e4) + sin(e2 + e3)*sin(e1)*sin(e4)) + cos(e6)*(cos(e5)*(cos(e1)*sin(e4) - sin(e2 + e3)*cos(e4)*sin(e1)) - cos(e2 + e3)*sin(e1)*sin(e5))))*(cos(e1)*(a1 + d4*cos(e2 + e3) + a3*sin(e2 + e3) + a2*sin(e2)) + x6*(sin(e6)*(cos(e4)*sin(e1) - sin(e2 + e3)*cos(e1)*sin(e4)) + cos(e6)*(cos(e5)*(sin(e1)*sin(e4) + sin(e2 + e3)*cos(e1)*cos(e4)) + cos(e2 + e3)*cos(e1)*sin(e5))) + y6*(cos(e6)*(cos(e4)*sin(e1) - sin(e2 + e3)*cos(e1)*sin(e4)) - sin(e6)*(cos(e5)*(sin(e1)*sin(e4) + sin(e2 + e3)*cos(e1)*cos(e4)) + cos(e2 + e3)*cos(e1)*sin(e5))) - z6*(sin(e5)*(sin(e1)*sin(e4) + sin(e2 + e3)*cos(e1)*cos(e4)) - cos(e2 + e3)*cos(e1)*cos(e5))) - m6*(x6*(cos(e6)*(cos(e4)*sin(e1) - sin(e2 + e3)*cos(e1)*sin(e4)) - sin(e6)*(cos(e5)*(sin(e1)*sin(e4) + sin(e2 + e3)*cos(e1)*cos(e4)) + cos(e2 + e3)*cos(e1)*sin(e5))) - y6*(sin(e6)*(cos(e4)*sin(e1) - sin(e2 + e3)*cos(e1)*sin(e4)) + cos(e6)*(cos(e5)*(sin(e1)*sin(e4) + sin(e2 + e3)*cos(e1)*cos(e4)) + cos(e2 + e3)*cos(e1)*sin(e5))))*(sin(e1)*(a1 + d4*cos(e2 + e3) + a3*sin(e2 + e3) + a2*sin(e2)) - x6*(sin(e6)*(cos(e1)*cos(e4) + sin(e2 + e3)*sin(e1)*sin(e4)) + cos(e6)*(cos(e5)*(cos(e1)*sin(e4) - sin(e2 + e3)*cos(e4)*sin(e1)) - cos(e2 + e3)*sin(e1)*sin(e5))) - y6*(cos(e6)*(cos(e1)*cos(e4) + sin(e2 + e3)*sin(e1)*sin(e4)) - sin(e6)*(cos(e5)*(cos(e1)*sin(e4) - sin(e2 + e3)*cos(e4)*sin(e1)) - cos(e2 + e3)*sin(e1)*sin(e5))) + z6*(sin(e5)*(cos(e1)*sin(e4) - sin(e2 + e3)*cos(e4)*sin(e1)) + cos(e2 + e3)*cos(e5)*sin(e1)));
 (I5zx*cos(e4) + I5xx*cos(e5)*sin(e4) + I5xy*sin(e4)*sin(e5))*(cos(e2)*sin(e3)*sin(e5) + cos(e3)*sin(e2)*sin(e5) - cos(e2)*cos(e3)*cos(e4)*cos(e5) + cos(e4)*cos(e5)*sin(e2)*sin(e3)) - (I5xy*cos(e5)*sin(e4) - I5yz*cos(e4) + I5yy*sin(e4)*sin(e5))*(cos(e2)*cos(e5)*sin(e3) + cos(e3)*cos(e5)*sin(e2) + cos(e2)*cos(e3)*cos(e4)*sin(e5) - cos(e4)*sin(e2)*sin(e3)*sin(e5)) - I3zx*cos(e2 + e3) + I3yz*sin(e2 + e3) - sin(e2 + e3)*(I4yz*cos(e4) + I4zx*sin(e4)) - I2zx*cos(e2) + (I6xx*(cos(e4)*sin(e6) + cos(e5)*cos(e6)*sin(e4)) - I6xy*(cos(e4)*cos(e6) - cos(e5)*sin(e4)*sin(e6)) + I6zx*sin(e4)*sin(e5))*(cos(e2)*cos(e3)*sin(e4)*sin(e6) + cos(e2)*cos(e6)*sin(e3)*sin(e5) + cos(e3)*cos(e6)*sin(e2)*sin(e5) - sin(e2)*sin(e3)*sin(e4)*sin(e6) - cos(e2)*cos(e3)*cos(e4)*cos(e5)*cos(e6) + cos(e4)*cos(e5)*cos(e6)*sin(e2)*sin(e3)) + I2yz*sin(e2) - (I6yy*(cos(e4)*cos(e6) - cos(e5)*sin(e4)*sin(e6)) - I6xy*(cos(e4)*sin(e6) + cos(e5)*cos(e6)*sin(e4)) + I6yz*sin(e4)*sin(e5))*(cos(e6)*sin(e2)*sin(e3)*sin(e4) - cos(e2)*cos(e3)*cos(e6)*sin(e4) + cos(e2)*sin(e3)*sin(e5)*sin(e6) + cos(e3)*sin(e2)*sin(e5)*sin(e6) - cos(e2)*cos(e3)*cos(e4)*cos(e5)*sin(e6) + cos(e4)*cos(e5)*sin(e2)*sin(e3)*sin(e6)) + (I4xy*cos(e4) - I4xx*sin(e4))*(cos(e2)*cos(e3)*cos(e4) - cos(e4)*sin(e2)*sin(e3)) + (cos(e2)*cos(e3)*sin(e4) - sin(e2)*sin(e3)*sin(e4))*(I4yy*cos(e4) - I4xy*sin(e4)) + (cos(e2)*cos(e3)*sin(e4) - sin(e2)*sin(e3)*sin(e4))*(I5zz*cos(e4) + I5zx*cos(e5)*sin(e4) - I5yz*sin(e4)*sin(e5)) - (I6yz*(cos(e4)*cos(e6) - cos(e5)*sin(e4)*sin(e6)) + I6zx*(cos(e4)*sin(e6) + cos(e5)*cos(e6)*sin(e4)) + I6zz*sin(e4)*sin(e5))*(cos(e2)*cos(e5)*sin(e3) + cos(e3)*cos(e5)*sin(e2) + cos(e2)*cos(e3)*cos(e4)*sin(e5) - cos(e4)*sin(e2)*sin(e3)*sin(e5)) - m3*(x3*cos(e2 + e3)*cos(e1) - y3*sin(e2 + e3)*cos(e1) + a2*cos(e1)*cos(e2))*(sin(e1)*(a1 + a2*sin(e2)) + z3*cos(e1) + y3*cos(e2 + e3)*sin(e1) + x3*sin(e2 + e3)*sin(e1)) + m3*(x3*cos(e2 + e3)*sin(e1) - y3*sin(e2 + e3)*sin(e1) + a2*cos(e2)*sin(e1))*(cos(e1)*(a1 + a2*sin(e2)) - z3*sin(e1) + y3*cos(e2 + e3)*cos(e1) + x3*sin(e2 + e3)*cos(e1)) + m6*(sin(e1)*(a1 + d4*cos(e2 + e3) + a3*sin(e2 + e3) + a2*sin(e2)) - x6*(sin(e6)*(cos(e1)*cos(e4) + sin(e2 + e3)*sin(e1)*sin(e4)) + cos(e6)*(cos(e5)*(cos(e1)*sin(e4) - sin(e2 + e3)*cos(e4)*sin(e1)) - cos(e2 + e3)*sin(e1)*sin(e5))) - y6*(cos(e6)*(cos(e1)*cos(e4) + sin(e2 + e3)*sin(e1)*sin(e4)) - sin(e6)*(cos(e5)*(cos(e1)*sin(e4) - sin(e2 + e3)*cos(e4)*sin(e1)) - cos(e2 + e3)*sin(e1)*sin(e5))) + z6*(sin(e5)*(cos(e1)*sin(e4) - sin(e2 + e3)*cos(e4)*sin(e1)) + cos(e2 + e3)*cos(e5)*sin(e1)))*(x6*(cos(e6)*(sin(e2 + e3)*cos(e1)*sin(e5) - cos(e2 + e3)*cos(e1)*cos(e4)*cos(e5)) + cos(e2 + e3)*cos(e1)*sin(e4)*sin(e6)) - y6*(sin(e6)*(sin(e2 + e3)*cos(e1)*sin(e5) - cos(e2 + e3)*cos(e1)*cos(e4)*cos(e5)) - cos(e2 + e3)*cos(e1)*cos(e6)*sin(e4)) + z6*(sin(e2 + e3)*cos(e1)*cos(e5) + cos(e2 + e3)*cos(e1)*cos(e4)*sin(e5)) - cos(e1)*(a3*cos(e2 + e3) - d4*sin(e2 + e3) + a2*cos(e2))) - m6*(cos(e1)*(a1 + d4*cos(e2 + e3) + a3*sin(e2 + e3) + a2*sin(e2)) + x6*(sin(e6)*(cos(e4)*sin(e1) - sin(e2 + e3)*cos(e1)*sin(e4)) + cos(e6)*(cos(e5)*(sin(e1)*sin(e4) + sin(e2 + e3)*cos(e1)*cos(e4)) + cos(e2 + e3)*cos(e1)*sin(e5))) + y6*(cos(e6)*(cos(e4)*sin(e1) - sin(e2 + e3)*cos(e1)*sin(e4)) - sin(e6)*(cos(e5)*(sin(e1)*sin(e4) + sin(e2 + e3)*cos(e1)*cos(e4)) + cos(e2 + e3)*cos(e1)*sin(e5))) - z6*(sin(e5)*(sin(e1)*sin(e4) + sin(e2 + e3)*cos(e1)*cos(e4)) - cos(e2 + e3)*cos(e1)*cos(e5)))*(x6*(cos(e6)*(sin(e2 + e3)*sin(e1)*sin(e5) - cos(e2 + e3)*cos(e4)*cos(e5)*sin(e1)) + cos(e2 + e3)*sin(e1)*sin(e4)*sin(e6)) - y6*(sin(e6)*(sin(e2 + e3)*sin(e1)*sin(e5) - cos(e2 + e3)*cos(e4)*cos(e5)*sin(e1)) - cos(e2 + e3)*cos(e6)*sin(e1)*sin(e4)) + z6*(sin(e2 + e3)*cos(e5)*sin(e1) + cos(e2 + e3)*cos(e4)*sin(e1)*sin(e5)) - sin(e1)*(a3*cos(e2 + e3) - d4*sin(e2 + e3) + a2*cos(e2))) + m5*(x5*(sin(e2 + e3)*cos(e1)*sin(e5) - cos(e2 + e3)*cos(e1)*cos(e4)*cos(e5)) + y5*(sin(e2 + e3)*cos(e1)*cos(e5) + cos(e2 + e3)*cos(e1)*cos(e4)*sin(e5)) - cos(e1)*(a3*cos(e2 + e3) - d4*sin(e2 + e3) + a2*cos(e2)) - z5*cos(e2 + e3)*cos(e1)*sin(e4))*(sin(e1)*(a1 + d4*cos(e2 + e3) + a3*sin(e2 + e3) + a2*sin(e2)) + z5*(cos(e1)*cos(e4) + sin(e2 + e3)*sin(e1)*sin(e4)) - x5*(cos(e5)*(cos(e1)*sin(e4) - sin(e2 + e3)*cos(e4)*sin(e1)) - cos(e2 + e3)*sin(e1)*sin(e5)) + y5*(sin(e5)*(cos(e1)*sin(e4) - sin(e2 + e3)*cos(e4)*sin(e1)) + cos(e2 + e3)*cos(e5)*sin(e1))) - m2*(x2*cos(e1)*cos(e2) - y2*cos(e1)*sin(e2))*(a1*sin(e1) + z2*cos(e1) + y2*cos(e2)*sin(e1) + x2*sin(e1)*sin(e2)) + m2*(x2*cos(e2)*sin(e1) - y2*sin(e1)*sin(e2))*(a1*cos(e1) - z2*sin(e1) + y2*cos(e1)*cos(e2) + x2*cos(e1)*sin(e2)) - m4*(cos(e1)*(a3*cos(e2 + e3) - d4*sin(e2 + e3) + a2*cos(e2)) - z4*sin(e2 + e3)*cos(e1) - y4*cos(e2 + e3)*cos(e1)*sin(e4) + x4*cos(e2 + e3)*cos(e1)*cos(e4))*(sin(e1)*(a1 + d4*cos(e2 + e3) + a3*sin(e2 + e3) + a2*sin(e2)) - x4*(cos(e1)*sin(e4) - sin(e2 + e3)*cos(e4)*sin(e1)) - y4*(cos(e1)*cos(e4) + sin(e2 + e3)*sin(e1)*sin(e4)) + z4*cos(e2 + e3)*sin(e1)) - m5*(cos(e1)*(a1 + d4*cos(e2 + e3) + a3*sin(e2 + e3) + a2*sin(e2)) - z5*(cos(e4)*sin(e1) - sin(e2 + e3)*cos(e1)*sin(e4)) + x5*(cos(e5)*(sin(e1)*sin(e4) + sin(e2 + e3)*cos(e1)*cos(e4)) + cos(e2 + e3)*cos(e1)*sin(e5)) - y5*(sin(e5)*(sin(e1)*sin(e4) + sin(e2 + e3)*cos(e1)*cos(e4)) - cos(e2 + e3)*cos(e1)*cos(e5)))*(x5*(sin(e2 + e3)*sin(e1)*sin(e5) - cos(e2 + e3)*cos(e4)*cos(e5)*sin(e1)) + y5*(sin(e2 + e3)*cos(e5)*sin(e1) + cos(e2 + e3)*cos(e4)*sin(e1)*sin(e5)) - sin(e1)*(a3*cos(e2 + e3) - d4*sin(e2 + e3) + a2*cos(e2)) - z5*cos(e2 + e3)*sin(e1)*sin(e4)) + m4*(cos(e1)*(a1 + d4*cos(e2 + e3) + a3*sin(e2 + e3) + a2*sin(e2)) + x4*(sin(e1)*sin(e4) + sin(e2 + e3)*cos(e1)*cos(e4)) + y4*(cos(e4)*sin(e1) - sin(e2 + e3)*cos(e1)*sin(e4)) + z4*cos(e2 + e3)*cos(e1))*(sin(e1)*(a3*cos(e2 + e3) - d4*sin(e2 + e3) + a2*cos(e2)) - z4*sin(e2 + e3)*sin(e1) + x4*cos(e2 + e3)*cos(e4)*sin(e1) - y4*cos(e2 + e3)*sin(e1)*sin(e4)),I4xx + I5yy + I2zz + I3zz + I6zz + a2^2*m3 + a2^2*m4 + a2^2*m5 + a3^2*m4 + a2^2*m6 + a3^2*m5 + a3^2*m6 + d4^2*m4 + d4^2*m5 + d4^2*m6 + m2*x2^2 + m3*x3^2 + m5*x5^2 + m6*x6^2 + m2*y2^2 + m3*y3^2 + m4*y4^2 + m6*y6^2 + m4*z4^2 + m5*z5^2 - I4xx*cos(e4)^2 + I5xx*cos(e5)^2 + I6xx*cos(e4)^2 + I4yy*cos(e4)^2 - I5yy*cos(e4)^2 - I5yy*cos(e5)^2 + I6yy*cos(e5)^2 + I5zz*cos(e4)^2 - I6zz*cos(e4)^2 - I6zz*cos(e5)^2 - I4xy*sin(2*e4) + I5xy*sin(2*e5) + 2*d4*m4*z4 + m4*x4^2*cos(e4)^2 - m5*x5^2*cos(e5)^2 - m6*x6^2*cos(e4)^2 - m4*y4^2*cos(e4)^2 + m5*y5^2*cos(e4)^2 + m5*y5^2*cos(e5)^2 - m6*y6^2*cos(e5)^2 - m5*z5^2*cos(e4)^2 + m6*z6^2*cos(e4)^2 + m6*z6^2*cos(e5)^2 - I5xx*cos(e4)^2*cos(e5)^2 - I6xx*cos(e4)^2*cos(e6)^2 + I6xx*cos(e5)^2*cos(e6)^2 + I5yy*cos(e4)^2*cos(e5)^2 - I6yy*cos(e4)^2*cos(e5)^2 + I6yy*cos(e4)^2*cos(e6)^2 - I6yy*cos(e5)^2*cos(e6)^2 + I6zz*cos(e4)^2*cos(e5)^2 + 2*I6xy*cos(e4)*cos(e5)*sin(e4) + 2*I5zx*cos(e4)*cos(e5)*sin(e4) + 2*I6zx*cos(e5)*cos(e6)*sin(e5) - I6xx*cos(e4)^2*cos(e5)^2*cos(e6)^2 + I6yy*cos(e4)^2*cos(e5)^2*cos(e6)^2 - 2*I5yz*cos(e4)*sin(e4)*sin(e5) - 2*I6yz*cos(e5)*sin(e5)*sin(e6) + 2*a2*a3*m4*cos(e3) + 2*a2*a3*m5*cos(e3) + 2*a2*a3*m6*cos(e3) - 2*a2*d4*m4*sin(e3) - 2*a2*d4*m5*sin(e3) - 2*a2*d4*m6*sin(e3) + 2*a2*m3*x3*cos(e3) + 2*a3*m4*x4*cos(e4) - 2*I5xy*cos(e4)^2*cos(e5)*sin(e5) - 2*I6xy*cos(e4)^2*cos(e6)*sin(e6) + 2*I6xy*cos(e5)^2*cos(e6)*sin(e6) + 2*d4*m5*y5*cos(e5) + 2*d4*m6*z6*cos(e5) - 2*a2*m3*y3*sin(e3) - 2*a3*m4*y4*sin(e4) - 2*a2*m4*z4*sin(e3) + 2*a3*m5*z5*sin(e4) + 2*d4*m5*x5*sin(e5) + m5*x5^2*cos(e4)^2*cos(e5)^2 + m6*x6^2*cos(e4)^2*cos(e6)^2 - m6*x6^2*cos(e5)^2*cos(e6)^2 - m5*y5^2*cos(e4)^2*cos(e5)^2 + m6*y6^2*cos(e4)^2*cos(e5)^2 - m6*y6^2*cos(e4)^2*cos(e6)^2 + m6*y6^2*cos(e5)^2*cos(e6)^2 - m4*x4*y4*sin(2*e4) + m5*x5*y5*sin(2*e5) - m6*z6^2*cos(e4)^2*cos(e5)^2 + m6*x6^2*cos(e4)^2*cos(e5)^2*cos(e6)^2 - m6*y6^2*cos(e4)^2*cos(e5)^2*cos(e6)^2 + 2*a2*m4*x4*cos(e3)*cos(e4) + 2*a3*m5*x5*cos(e4)*cos(e5) - 4*I6xy*cos(e4)*cos(e5)*cos(e6)^2*sin(e4) - 2*I6zx*cos(e4)^2*cos(e5)*cos(e6)*sin(e5) - 2*a2*m4*y4*cos(e3)*sin(e4) - 2*a2*m5*y5*cos(e5)*sin(e3) - 2*a3*m5*y5*cos(e4)*sin(e5) - 2*a3*m6*y6*cos(e6)*sin(e4) + 2*a2*m5*z5*cos(e3)*sin(e4) - 2*a2*m6*z6*cos(e5)*sin(e3) - 2*a3*m6*z6*cos(e4)*sin(e5) + 2*d4*m6*x6*cos(e6)*sin(e5) + 2*I6yz*cos(e4)^2*cos(e5)*sin(e5)*sin(e6) - 2*a2*m5*x5*sin(e3)*sin(e5) - 2*a3*m6*x6*sin(e4)*sin(e6) - 2*d4*m6*y6*sin(e5)*sin(e6) - 2*I6xy*cos(e4)^2*cos(e5)^2*cos(e6)*sin(e6) + 2*I6yz*cos(e4)*cos(e6)*sin(e4)*sin(e5) + 2*I6zx*cos(e4)*sin(e4)*sin(e5)*sin(e6) - 2*a2*m5*y5*cos(e3)*cos(e4)*sin(e5) - 2*a2*m6*y6*cos(e3)*cos(e6)*sin(e4) - 2*a3*m6*y6*cos(e4)*cos(e5)*sin(e6) - 2*a2*m6*z6*cos(e3)*cos(e4)*sin(e5) - 2*a2*m6*x6*cos(e3)*sin(e4)*sin(e6) - 2*a2*m6*x6*cos(e6)*sin(e3)*sin(e5) + 2*m6*x6*y6*cos(e4)*cos(e5)*sin(e4) + 2*m5*x5*z5*cos(e4)*cos(e5)*sin(e4) + 2*m6*x6*z6*cos(e5)*cos(e6)*sin(e5) + 2*a2*m6*y6*sin(e3)*sin(e5)*sin(e6) - 2*m5*y5*z5*cos(e4)*sin(e4)*sin(e5) - 2*m6*y6*z6*cos(e5)*sin(e5)*sin(e6) - 2*m5*x5*y5*cos(e4)^2*cos(e5)*sin(e5) - 2*m6*x6*y6*cos(e4)^2*cos(e6)*sin(e6) + 2*m6*x6*y6*cos(e5)^2*cos(e6)*sin(e6) + 2*I6xx*cos(e4)*cos(e5)*cos(e6)*sin(e4)*sin(e6) - 2*I6yy*cos(e4)*cos(e5)*cos(e6)*sin(e4)*sin(e6) + 2*a2*m5*x5*cos(e3)*cos(e4)*cos(e5) + 2*a3*m6*x6*cos(e4)*cos(e5)*cos(e6) + 2*m6*y6*z6*cos(e4)*cos(e6)*sin(e4)*sin(e5) + 2*m6*x6*z6*cos(e4)*sin(e4)*sin(e5)*sin(e6) - 4*m6*x6*y6*cos(e4)*cos(e5)*cos(e6)^2*sin(e4) - 2*m6*x6*z6*cos(e4)^2*cos(e5)*cos(e6)*sin(e5) + 2*m6*y6*z6*cos(e4)^2*cos(e5)*sin(e5)*sin(e6) - 2*m6*x6^2*cos(e4)*cos(e5)*cos(e6)*sin(e4)*sin(e6) - 2*m6*x6*y6*cos(e4)^2*cos(e5)^2*cos(e6)*sin(e6) + 2*m6*y6^2*cos(e4)*cos(e5)*cos(e6)*sin(e4)*sin(e6) + 2*a2*m6*x6*cos(e3)*cos(e4)*cos(e5)*cos(e6) - 2*a2*m6*y6*cos(e3)*cos(e4)*cos(e5)*sin(e6),I4xx + I5yy + I3zz + I6zz + a3^2*m4 + a3^2*m5 + a3^2*m6 + d4^2*m4 + d4^2*m5 + d4^2*m6 + m3*x3^2 + m5*x5^2 + m6*x6^2 + m3*y3^2 + m4*y4^2 + m6*y6^2 + m4*z4^2 + m5*z5^2 - I4xx*cos(e4)^2 + I5xx*cos(e5)^2 + I6xx*cos(e4)^2 + I4yy*cos(e4)^2 - I5yy*cos(e4)^2 - I5yy*cos(e5)^2 + I6yy*cos(e5)^2 + I5zz*cos(e4)^2 - I6zz*cos(e4)^2 - I6zz*cos(e5)^2 - I4xy*sin(2*e4) + I5xy*sin(2*e5) + 2*d4*m4*z4 + m4*x4^2*cos(e4)^2 - m5*x5^2*cos(e5)^2 - m6*x6^2*cos(e4)^2 - m4*y4^2*cos(e4)^2 + m5*y5^2*cos(e4)^2 + m5*y5^2*cos(e5)^2 - m6*y6^2*cos(e5)^2 - m5*z5^2*cos(e4)^2 + m6*z6^2*cos(e4)^2 + m6*z6^2*cos(e5)^2 - I5xx*cos(e4)^2*cos(e5)^2 - I6xx*cos(e4)^2*cos(e6)^2 + I6xx*cos(e5)^2*cos(e6)^2 + I5yy*cos(e4)^2*cos(e5)^2 - I6yy*cos(e4)^2*cos(e5)^2 + I6yy*cos(e4)^2*cos(e6)^2 - I6yy*cos(e5)^2*cos(e6)^2 + I6zz*cos(e4)^2*cos(e5)^2 + 2*I6xy*cos(e4)*cos(e5)*sin(e4) + 2*I5zx*cos(e4)*cos(e5)*sin(e4) + 2*I6zx*cos(e5)*cos(e6)*sin(e5) - I6xx*cos(e4)^2*cos(e5)^2*cos(e6)^2 + I6yy*cos(e4)^2*cos(e5)^2*cos(e6)^2 - 2*I5yz*cos(e4)*sin(e4)*sin(e5) - 2*I6yz*cos(e5)*sin(e5)*sin(e6) + a2*a3*m4*cos(e3) + a2*a3*m5*cos(e3) + a2*a3*m6*cos(e3) - a2*d4*m4*sin(e3) - a2*d4*m5*sin(e3) - a2*d4*m6*sin(e3) + a2*m3*x3*cos(e3) + 2*a3*m4*x4*cos(e4) - 2*I5xy*cos(e4)^2*cos(e5)*sin(e5) - 2*I6xy*cos(e4)^2*cos(e6)*sin(e6) + 2*I6xy*cos(e5)^2*cos(e6)*sin(e6) + 2*d4*m5*y5*cos(e5) + 2*d4*m6*z6*cos(e5) - a2*m3*y3*sin(e3) - 2*a3*m4*y4*sin(e4) - a2*m4*z4*sin(e3) + 2*a3*m5*z5*sin(e4) + 2*d4*m5*x5*sin(e5) + m5*x5^2*cos(e4)^2*cos(e5)^2 + m6*x6^2*cos(e4)^2*cos(e6)^2 - m6*x6^2*cos(e5)^2*cos(e6)^2 - m5*y5^2*cos(e4)^2*cos(e5)^2 + m6*y6^2*cos(e4)^2*cos(e5)^2 - m6*y6^2*cos(e4)^2*cos(e6)^2 + m6*y6^2*cos(e5)^2*cos(e6)^2 - m4*x4*y4*sin(2*e4) + m5*x5*y5*sin(2*e5) - m6*z6^2*cos(e4)^2*cos(e5)^2 + m6*x6^2*cos(e4)^2*cos(e5)^2*cos(e6)^2 - m6*y6^2*cos(e4)^2*cos(e5)^2*cos(e6)^2 + a2*m4*x4*cos(e3)*cos(e4) + 2*a3*m5*x5*cos(e4)*cos(e5) - 4*I6xy*cos(e4)*cos(e5)*cos(e6)^2*sin(e4) - 2*I6zx*cos(e4)^2*cos(e5)*cos(e6)*sin(e5) - a2*m4*y4*cos(e3)*sin(e4) - a2*m5*y5*cos(e5)*sin(e3) - 2*a3*m5*y5*cos(e4)*sin(e5) - 2*a3*m6*y6*cos(e6)*sin(e4) + a2*m5*z5*cos(e3)*sin(e4) - a2*m6*z6*cos(e5)*sin(e3) - 2*a3*m6*z6*cos(e4)*sin(e5) + 2*d4*m6*x6*cos(e6)*sin(e5) + 2*I6yz*cos(e4)^2*cos(e5)*sin(e5)*sin(e6) - a2*m5*x5*sin(e3)*sin(e5) - 2*a3*m6*x6*sin(e4)*sin(e6) - 2*d4*m6*y6*sin(e5)*sin(e6) - 2*I6xy*cos(e4)^2*cos(e5)^2*cos(e6)*sin(e6) + 2*I6yz*cos(e4)*cos(e6)*sin(e4)*sin(e5) + 2*I6zx*cos(e4)*sin(e4)*sin(e5)*sin(e6) - a2*m5*y5*cos(e3)*cos(e4)*sin(e5) - a2*m6*y6*cos(e3)*cos(e6)*sin(e4) - 2*a3*m6*y6*cos(e4)*cos(e5)*sin(e6) - a2*m6*z6*cos(e3)*cos(e4)*sin(e5) - a2*m6*x6*cos(e3)*sin(e4)*sin(e6) - a2*m6*x6*cos(e6)*sin(e3)*sin(e5) + 2*m6*x6*y6*cos(e4)*cos(e5)*sin(e4) + 2*m5*x5*z5*cos(e4)*cos(e5)*sin(e4) + 2*m6*x6*z6*cos(e5)*cos(e6)*sin(e5) + a2*m6*y6*sin(e3)*sin(e5)*sin(e6) - 2*m5*y5*z5*cos(e4)*sin(e4)*sin(e5) - 2*m6*y6*z6*cos(e5)*sin(e5)*sin(e6) - 2*m5*x5*y5*cos(e4)^2*cos(e5)*sin(e5) - 2*m6*x6*y6*cos(e4)^2*cos(e6)*sin(e6) + 2*m6*x6*y6*cos(e5)^2*cos(e6)*sin(e6) + 2*I6xx*cos(e4)*cos(e5)*cos(e6)*sin(e4)*sin(e6) - 2*I6yy*cos(e4)*cos(e5)*cos(e6)*sin(e4)*sin(e6) + a2*m5*x5*cos(e3)*cos(e4)*cos(e5) + 2*a3*m6*x6*cos(e4)*cos(e5)*cos(e6) + 2*m6*y6*z6*cos(e4)*cos(e6)*sin(e4)*sin(e5) + 2*m6*x6*z6*cos(e4)*sin(e4)*sin(e5)*sin(e6) - 4*m6*x6*y6*cos(e4)*cos(e5)*cos(e6)^2*sin(e4) - 2*m6*x6*z6*cos(e4)^2*cos(e5)*cos(e6)*sin(e5) + 2*m6*y6*z6*cos(e4)^2*cos(e5)*sin(e5)*sin(e6) - 2*m6*x6^2*cos(e4)*cos(e5)*cos(e6)*sin(e4)*sin(e6) - 2*m6*x6*y6*cos(e4)^2*cos(e5)^2*cos(e6)*sin(e6) + 2*m6*y6^2*cos(e4)*cos(e5)*cos(e6)*sin(e4)*sin(e6) + a2*m6*x6*cos(e3)*cos(e4)*cos(e5)*cos(e6) - a2*m6*y6*cos(e3)*cos(e4)*cos(e5)*sin(e6),I4yz*cos(e4) - I5xy*sin(e4) + I4zx*sin(e4) - I5yz*cos(e4)*cos(e5) - I6xy*cos(e4)*sin(e5) - I5zx*cos(e4)*sin(e5) - I6zx*cos(e6)*sin(e4) + I6yz*sin(e4)*sin(e6) + 2*I5xy*cos(e5)^2*sin(e4) + I6yz*cos(e4)*cos(e5)*cos(e6) + I6zx*cos(e4)*cos(e5)*sin(e6) - I5xx*cos(e5)*sin(e4)*sin(e5) + I5yy*cos(e5)*sin(e4)*sin(e5) - I6yy*cos(e5)*sin(e4)*sin(e5) + I6zz*cos(e5)*sin(e4)*sin(e5) + 2*I6xy*cos(e4)*cos(e6)^2*sin(e5) + 2*I6zx*cos(e5)^2*cos(e6)*sin(e4) + d4*m4*y4*cos(e4) - d4*m5*z5*cos(e4) + d4*m4*x4*sin(e4) - 2*I6yz*cos(e5)^2*sin(e4)*sin(e6) + m4*y4*z4*cos(e4) - m5*x5*y5*sin(e4) + m4*x4*z4*sin(e4) + m5*x5^2*cos(e5)*sin(e4)*sin(e5) - m5*y5^2*cos(e5)*sin(e4)*sin(e5) + m6*y6^2*cos(e5)*sin(e4)*sin(e5) - m6*z6^2*cos(e5)*sin(e4)*sin(e5) + d4*m6*y6*cos(e4)*cos(e6) - a2*m4*y4*cos(e4)*sin(e3) + a2*m5*z5*cos(e4)*sin(e3) + d4*m5*x5*cos(e5)*sin(e4) + d4*m6*x6*cos(e4)*sin(e6) - I6xx*cos(e5)*cos(e6)^2*sin(e4)*sin(e5) + I6yy*cos(e5)*cos(e6)^2*sin(e4)*sin(e5) - m5*y5*z5*cos(e4)*cos(e5) - a2*m4*x4*sin(e3)*sin(e4) - d4*m5*y5*sin(e4)*sin(e5) - d4*m6*z6*sin(e4)*sin(e5) - m6*x6*y6*cos(e4)*sin(e5) - m5*x5*z5*cos(e4)*sin(e5) - m6*x6*z6*cos(e6)*sin(e4) + m6*y6*z6*sin(e4)*sin(e6) + 2*m5*x5*y5*cos(e5)^2*sin(e4) - I6xx*cos(e4)*cos(e6)*sin(e5)*sin(e6) + I6yy*cos(e4)*cos(e6)*sin(e5)*sin(e6) - a2*m6*y6*cos(e4)*cos(e6)*sin(e3) + d4*m6*x6*cos(e5)*cos(e6)*sin(e4) + m6*y6*z6*cos(e4)*cos(e5)*cos(e6) - a2*m5*x5*cos(e5)*sin(e3)*sin(e4) - a2*m6*x6*cos(e4)*sin(e3)*sin(e6) - d4*m6*y6*cos(e5)*sin(e4)*sin(e6) + m6*x6*z6*cos(e4)*cos(e5)*sin(e6) + a2*m5*y5*sin(e3)*sin(e4)*sin(e5) + a2*m6*z6*sin(e3)*sin(e4)*sin(e5) + m6*x6^2*cos(e5)*cos(e6)^2*sin(e4)*sin(e5) - m6*y6^2*cos(e5)*cos(e6)^2*sin(e4)*sin(e5) + 2*m6*x6*y6*cos(e4)*cos(e6)^2*sin(e5) + 2*m6*x6*z6*cos(e5)^2*cos(e6)*sin(e4) - 2*m6*y6*z6*cos(e5)^2*sin(e4)*sin(e6) - 2*I6xy*cos(e5)*cos(e6)*sin(e4)*sin(e5)*sin(e6) + m6*x6^2*cos(e4)*cos(e6)*sin(e5)*sin(e6) - m6*y6^2*cos(e4)*cos(e6)*sin(e5)*sin(e6) - a2*m6*x6*cos(e5)*cos(e6)*sin(e3)*sin(e4) + a2*m6*y6*cos(e5)*sin(e3)*sin(e4)*sin(e6) - 2*m6*x6*y6*cos(e5)*cos(e6)*sin(e4)*sin(e5)*sin(e6),I6xx*cos(e4) + I5zz*cos(e4) + I6xy*cos(e5)*sin(e4) + I5zx*cos(e5)*sin(e4) - I5yz*sin(e4)*sin(e5) + m5*x5^2*cos(e4) + m5*y5^2*cos(e4) + m6*y6^2*cos(e4) + m6*z6^2*cos(e4) - I6xx*cos(e4)*cos(e6)^2 + I6yy*cos(e4)*cos(e6)^2 - 2*I6xy*cos(e4)*cos(e6)*sin(e6) + I6yz*cos(e6)*sin(e4)*sin(e5) + I6zx*sin(e4)*sin(e5)*sin(e6) + a3*m5*x5*cos(e5) - 2*I6xy*cos(e5)*cos(e6)^2*sin(e4) - a3*m5*y5*sin(e5) - a3*m6*z6*sin(e5) + m6*x6^2*cos(e4)*cos(e6)^2 - m6*y6^2*cos(e4)*cos(e6)^2 + a2*m5*x5*cos(e3)*cos(e5) + a3*m6*x6*cos(e5)*cos(e6) + d4*m5*y5*cos(e4)*cos(e5) + d4*m6*z6*cos(e4)*cos(e5) - a2*m5*y5*cos(e3)*sin(e5) - a3*m6*y6*cos(e5)*sin(e6) - a2*m6*z6*cos(e3)*sin(e5) + d4*m5*x5*cos(e4)*sin(e5) + m6*x6*y6*cos(e5)*sin(e4) + m5*x5*z5*cos(e5)*sin(e4) - m5*y5*z5*sin(e4)*sin(e5) + I6xx*cos(e5)*cos(e6)*sin(e4)*sin(e6) - I6yy*cos(e5)*cos(e6)*sin(e4)*sin(e6) - a2*m5*y5*cos(e4)*cos(e5)*sin(e3) - a2*m6*y6*cos(e3)*cos(e5)*sin(e6) - a2*m6*z6*cos(e4)*cos(e5)*sin(e3) + d4*m6*x6*cos(e4)*cos(e6)*sin(e5) - a2*m5*x5*cos(e4)*sin(e3)*sin(e5) - d4*m6*y6*cos(e4)*sin(e5)*sin(e6) - 2*m6*x6*y6*cos(e4)*cos(e6)*sin(e6) + m6*y6*z6*cos(e6)*sin(e4)*sin(e5) + m6*x6*z6*sin(e4)*sin(e5)*sin(e6) - 2*m6*x6*y6*cos(e5)*cos(e6)^2*sin(e4) - m6*x6^2*cos(e5)*cos(e6)*sin(e4)*sin(e6) + m6*y6^2*cos(e5)*cos(e6)*sin(e4)*sin(e6) + a2*m6*x6*cos(e3)*cos(e5)*cos(e6) - a2*m6*x6*cos(e4)*cos(e6)*sin(e3)*sin(e5) + a2*m6*y6*cos(e4)*sin(e3)*sin(e5)*sin(e6),I6yz*cos(e4)*cos(e6) + I6zx*cos(e4)*sin(e6) + I6zz*sin(e4)*sin(e5) + I6zx*cos(e5)*cos(e6)*sin(e4) - I6yz*cos(e5)*sin(e4)*sin(e6) + m6*x6^2*sin(e4)*sin(e5) + m6*y6^2*sin(e4)*sin(e5) - a3*m6*y6*cos(e6)*sin(e5) + d4*m6*x6*cos(e6)*sin(e4) + m6*y6*z6*cos(e4)*cos(e6) - a3*m6*x6*sin(e5)*sin(e6) - d4*m6*y6*sin(e4)*sin(e6) + m6*x6*z6*cos(e4)*sin(e6) + d4*m6*y6*cos(e4)*cos(e5)*cos(e6) - a2*m6*y6*cos(e3)*cos(e6)*sin(e5) + d4*m6*x6*cos(e4)*cos(e5)*sin(e6) - a2*m6*x6*cos(e6)*sin(e3)*sin(e4) - a2*m6*x6*cos(e3)*sin(e5)*sin(e6) + m6*x6*z6*cos(e5)*cos(e6)*sin(e4) + a2*m6*y6*sin(e3)*sin(e4)*sin(e6) - m6*y6*z6*cos(e5)*sin(e4)*sin(e6) - a2*m6*y6*cos(e4)*cos(e5)*cos(e6)*sin(e3) - a2*m6*x6*cos(e4)*cos(e5)*sin(e3)*sin(e6);
 (I5zx*cos(e4) + I5xx*cos(e5)*sin(e4) + I5xy*sin(e4)*sin(e5))*(cos(e2)*sin(e3)*sin(e5) + cos(e3)*sin(e2)*sin(e5) - cos(e2)*cos(e3)*cos(e4)*cos(e5) + cos(e4)*cos(e5)*sin(e2)*sin(e3)) - (I5xy*cos(e5)*sin(e4) - I5yz*cos(e4) + I5yy*sin(e4)*sin(e5))*(cos(e2)*cos(e5)*sin(e3) + cos(e3)*cos(e5)*sin(e2) + cos(e2)*cos(e3)*cos(e4)*sin(e5) - cos(e4)*sin(e2)*sin(e3)*sin(e5)) - I3zx*cos(e2 + e3) + I3yz*sin(e2 + e3) - sin(e2 + e3)*(I4yz*cos(e4) + I4zx*sin(e4)) + (I6xx*(cos(e4)*sin(e6) + cos(e5)*cos(e6)*sin(e4)) - I6xy*(cos(e4)*cos(e6) - cos(e5)*sin(e4)*sin(e6)) + I6zx*sin(e4)*sin(e5))*(cos(e2)*cos(e3)*sin(e4)*sin(e6) + cos(e2)*cos(e6)*sin(e3)*sin(e5) + cos(e3)*cos(e6)*sin(e2)*sin(e5) - sin(e2)*sin(e3)*sin(e4)*sin(e6) - cos(e2)*cos(e3)*cos(e4)*cos(e5)*cos(e6) + cos(e4)*cos(e5)*cos(e6)*sin(e2)*sin(e3)) - (I6yy*(cos(e4)*cos(e6) - cos(e5)*sin(e4)*sin(e6)) - I6xy*(cos(e4)*sin(e6) + cos(e5)*cos(e6)*sin(e4)) + I6yz*sin(e4)*sin(e5))*(cos(e6)*sin(e2)*sin(e3)*sin(e4) - cos(e2)*cos(e3)*cos(e6)*sin(e4) + cos(e2)*sin(e3)*sin(e5)*sin(e6) + cos(e3)*sin(e2)*sin(e5)*sin(e6) - cos(e2)*cos(e3)*cos(e4)*cos(e5)*sin(e6) + cos(e4)*cos(e5)*sin(e2)*sin(e3)*sin(e6)) + (I4xy*cos(e4) - I4xx*sin(e4))*(cos(e2)*cos(e3)*cos(e4) - cos(e4)*sin(e2)*sin(e3)) + (cos(e2)*cos(e3)*sin(e4) - sin(e2)*sin(e3)*sin(e4))*(I4yy*cos(e4) - I4xy*sin(e4)) + (cos(e2)*cos(e3)*sin(e4) - sin(e2)*sin(e3)*sin(e4))*(I5zz*cos(e4) + I5zx*cos(e5)*sin(e4) - I5yz*sin(e4)*sin(e5)) - (I6yz*(cos(e4)*cos(e6) - cos(e5)*sin(e4)*sin(e6)) + I6zx*(cos(e4)*sin(e6) + cos(e5)*cos(e6)*sin(e4)) + I6zz*sin(e4)*sin(e5))*(cos(e2)*cos(e5)*sin(e3) + cos(e3)*cos(e5)*sin(e2) + cos(e2)*cos(e3)*cos(e4)*sin(e5) - cos(e4)*sin(e2)*sin(e3)*sin(e5)) + m5*(sin(e1)*(a1 + d4*cos(e2 + e3) + a3*sin(e2 + e3) + a2*sin(e2)) + z5*(cos(e1)*cos(e4) + sin(e2 + e3)*sin(e1)*sin(e4)) - x5*(cos(e5)*(cos(e1)*sin(e4) - sin(e2 + e3)*cos(e4)*sin(e1)) - cos(e2 + e3)*sin(e1)*sin(e5)) + y5*(sin(e5)*(cos(e1)*sin(e4) - sin(e2 + e3)*cos(e4)*sin(e1)) + cos(e2 + e3)*cos(e5)*sin(e1)))*(x5*(sin(e2 + e3)*cos(e1)*sin(e5) - cos(e2 + e3)*cos(e1)*cos(e4)*cos(e5)) + y5*(sin(e2 + e3)*cos(e1)*cos(e5) + cos(e2 + e3)*cos(e1)*cos(e4)*sin(e5)) - cos(e1)*(a3*cos(e2 + e3) - d4*sin(e2 + e3)) - z5*cos(e2 + e3)*cos(e1)*sin(e4)) - m4*(sin(e1)*(a1 + d4*cos(e2 + e3) + a3*sin(e2 + e3) + a2*sin(e2)) - x4*(cos(e1)*sin(e4) - sin(e2 + e3)*cos(e4)*sin(e1)) - y4*(cos(e1)*cos(e4) + sin(e2 + e3)*sin(e1)*sin(e4)) + z4*cos(e2 + e3)*sin(e1))*(cos(e1)*(a3*cos(e2 + e3) - d4*sin(e2 + e3)) - z4*sin(e2 + e3)*cos(e1) - y4*cos(e2 + e3)*cos(e1)*sin(e4) + x4*cos(e2 + e3)*cos(e1)*cos(e4)) - m5*(x5*(sin(e2 + e3)*sin(e1)*sin(e5) - cos(e2 + e3)*cos(e4)*cos(e5)*sin(e1)) + y5*(sin(e2 + e3)*cos(e5)*sin(e1) + cos(e2 + e3)*cos(e4)*sin(e1)*sin(e5)) - sin(e1)*(a3*cos(e2 + e3) - d4*sin(e2 + e3)) - z5*cos(e2 + e3)*sin(e1)*sin(e4))*(cos(e1)*(a1 + d4*cos(e2 + e3) + a3*sin(e2 + e3) + a2*sin(e2)) - z5*(cos(e4)*sin(e1) - sin(e2 + e3)*cos(e1)*sin(e4)) + x5*(cos(e5)*(sin(e1)*sin(e4) + sin(e2 + e3)*cos(e1)*cos(e4)) + cos(e2 + e3)*cos(e1)*sin(e5)) - y5*(sin(e5)*(sin(e1)*sin(e4) + sin(e2 + e3)*cos(e1)*cos(e4)) - cos(e2 + e3)*cos(e1)*cos(e5))) + m4*(sin(e1)*(a3*cos(e2 + e3) - d4*sin(e2 + e3)) - z4*sin(e2 + e3)*sin(e1) + x4*cos(e2 + e3)*cos(e4)*sin(e1) - y4*cos(e2 + e3)*sin(e1)*sin(e4))*(cos(e1)*(a1 + d4*cos(e2 + e3) + a3*sin(e2 + e3) + a2*sin(e2)) + x4*(sin(e1)*sin(e4) + sin(e2 + e3)*cos(e1)*cos(e4)) + y4*(cos(e4)*sin(e1) - sin(e2 + e3)*cos(e1)*sin(e4)) + z4*cos(e2 + e3)*cos(e1)) + m6*(sin(e1)*(a1 + d4*cos(e2 + e3) + a3*sin(e2 + e3) + a2*sin(e2)) - x6*(sin(e6)*(cos(e1)*cos(e4) + sin(e2 + e3)*sin(e1)*sin(e4)) + cos(e6)*(cos(e5)*(cos(e1)*sin(e4) - sin(e2 + e3)*cos(e4)*sin(e1)) - cos(e2 + e3)*sin(e1)*sin(e5))) - y6*(cos(e6)*(cos(e1)*cos(e4) + sin(e2 + e3)*sin(e1)*sin(e4)) - sin(e6)*(cos(e5)*(cos(e1)*sin(e4) - sin(e2 + e3)*cos(e4)*sin(e1)) - cos(e2 + e3)*sin(e1)*sin(e5))) + z6*(sin(e5)*(cos(e1)*sin(e4) - sin(e2 + e3)*cos(e4)*sin(e1)) + cos(e2 + e3)*cos(e5)*sin(e1)))*(x6*(cos(e6)*(sin(e2 + e3)*cos(e1)*sin(e5) - cos(e2 + e3)*cos(e1)*cos(e4)*cos(e5)) + cos(e2 + e3)*cos(e1)*sin(e4)*sin(e6)) - y6*(sin(e6)*(sin(e2 + e3)*cos(e1)*sin(e5) - cos(e2 + e3)*cos(e1)*cos(e4)*cos(e5)) - cos(e2 + e3)*cos(e1)*cos(e6)*sin(e4)) + z6*(sin(e2 + e3)*cos(e1)*cos(e5) + cos(e2 + e3)*cos(e1)*cos(e4)*sin(e5)) - cos(e1)*(a3*cos(e2 + e3) - d4*sin(e2 + e3))) - m3*(x3*cos(e2 + e3)*cos(e1) - y3*sin(e2 + e3)*cos(e1))*(sin(e1)*(a1 + a2*sin(e2)) + z3*cos(e1) + y3*cos(e2 + e3)*sin(e1) + x3*sin(e2 + e3)*sin(e1)) + m3*(x3*cos(e2 + e3)*sin(e1) - y3*sin(e2 + e3)*sin(e1))*(cos(e1)*(a1 + a2*sin(e2)) - z3*sin(e1) + y3*cos(e2 + e3)*cos(e1) + x3*sin(e2 + e3)*cos(e1)) - m6*(x6*(cos(e6)*(sin(e2 + e3)*sin(e1)*sin(e5) - cos(e2 + e3)*cos(e4)*cos(e5)*sin(e1)) + cos(e2 + e3)*sin(e1)*sin(e4)*sin(e6)) - y6*(sin(e6)*(sin(e2 + e3)*sin(e1)*sin(e5) - cos(e2 + e3)*cos(e4)*cos(e5)*sin(e1)) - cos(e2 + e3)*cos(e6)*sin(e1)*sin(e4)) + z6*(sin(e2 + e3)*cos(e5)*sin(e1) + cos(e2 + e3)*cos(e4)*sin(e1)*sin(e5)) - sin(e1)*(a3*cos(e2 + e3) - d4*sin(e2 + e3)))*(cos(e1)*(a1 + d4*cos(e2 + e3) + a3*sin(e2 + e3) + a2*sin(e2)) + x6*(sin(e6)*(cos(e4)*sin(e1) - sin(e2 + e3)*cos(e1)*sin(e4)) + cos(e6)*(cos(e5)*(sin(e1)*sin(e4) + sin(e2 + e3)*cos(e1)*cos(e4)) + cos(e2 + e3)*cos(e1)*sin(e5))) + y6*(cos(e6)*(cos(e4)*sin(e1) - sin(e2 + e3)*cos(e1)*sin(e4)) - sin(e6)*(cos(e5)*(sin(e1)*sin(e4) + sin(e2 + e3)*cos(e1)*cos(e4)) + cos(e2 + e3)*cos(e1)*sin(e5))) - z6*(sin(e5)*(sin(e1)*sin(e4) + sin(e2 + e3)*cos(e1)*cos(e4)) - cos(e2 + e3)*cos(e1)*cos(e5))),I4xx + I5yy + I3zz + I6zz + a3^2*m4 + a3^2*m5 + a3^2*m6 + d4^2*m4 + d4^2*m5 + d4^2*m6 + m3*x3^2 + m5*x5^2 + m6*x6^2 + m3*y3^2 + m4*y4^2 + m6*y6^2 + m4*z4^2 + m5*z5^2 - I4xx*cos(e4)^2 + I5xx*cos(e5)^2 + I6xx*cos(e4)^2 + I4yy*cos(e4)^2 - I5yy*cos(e4)^2 - I5yy*cos(e5)^2 + I6yy*cos(e5)^2 + I5zz*cos(e4)^2 - I6zz*cos(e4)^2 - I6zz*cos(e5)^2 - I4xy*sin(2*e4) + I5xy*sin(2*e5) + 2*d4*m4*z4 + m4*x4^2*cos(e4)^2 - m5*x5^2*cos(e5)^2 - m6*x6^2*cos(e4)^2 - m4*y4^2*cos(e4)^2 + m5*y5^2*cos(e4)^2 + m5*y5^2*cos(e5)^2 - m6*y6^2*cos(e5)^2 - m5*z5^2*cos(e4)^2 + m6*z6^2*cos(e4)^2 + m6*z6^2*cos(e5)^2 - I5xx*cos(e4)^2*cos(e5)^2 - I6xx*cos(e4)^2*cos(e6)^2 + I6xx*cos(e5)^2*cos(e6)^2 + I5yy*cos(e4)^2*cos(e5)^2 - I6yy*cos(e4)^2*cos(e5)^2 + I6yy*cos(e4)^2*cos(e6)^2 - I6yy*cos(e5)^2*cos(e6)^2 + I6zz*cos(e4)^2*cos(e5)^2 + 2*I6xy*cos(e4)*cos(e5)*sin(e4) + 2*I5zx*cos(e4)*cos(e5)*sin(e4) + 2*I6zx*cos(e5)*cos(e6)*sin(e5) - I6xx*cos(e4)^2*cos(e5)^2*cos(e6)^2 + I6yy*cos(e4)^2*cos(e5)^2*cos(e6)^2 - 2*I5yz*cos(e4)*sin(e4)*sin(e5) - 2*I6yz*cos(e5)*sin(e5)*sin(e6) + a2*a3*m4*cos(e3) + a2*a3*m5*cos(e3) + a2*a3*m6*cos(e3) - a2*d4*m4*sin(e3) - a2*d4*m5*sin(e3) - a2*d4*m6*sin(e3) + a2*m3*x3*cos(e3) + 2*a3*m4*x4*cos(e4) - 2*I5xy*cos(e4)^2*cos(e5)*sin(e5) - 2*I6xy*cos(e4)^2*cos(e6)*sin(e6) + 2*I6xy*cos(e5)^2*cos(e6)*sin(e6) + 2*d4*m5*y5*cos(e5) + 2*d4*m6*z6*cos(e5) - a2*m3*y3*sin(e3) - 2*a3*m4*y4*sin(e4) - a2*m4*z4*sin(e3) + 2*a3*m5*z5*sin(e4) + 2*d4*m5*x5*sin(e5) + m5*x5^2*cos(e4)^2*cos(e5)^2 + m6*x6^2*cos(e4)^2*cos(e6)^2 - m6*x6^2*cos(e5)^2*cos(e6)^2 - m5*y5^2*cos(e4)^2*cos(e5)^2 + m6*y6^2*cos(e4)^2*cos(e5)^2 - m6*y6^2*cos(e4)^2*cos(e6)^2 + m6*y6^2*cos(e5)^2*cos(e6)^2 - m4*x4*y4*sin(2*e4) + m5*x5*y5*sin(2*e5) - m6*z6^2*cos(e4)^2*cos(e5)^2 + m6*x6^2*cos(e4)^2*cos(e5)^2*cos(e6)^2 - m6*y6^2*cos(e4)^2*cos(e5)^2*cos(e6)^2 + a2*m4*x4*cos(e3)*cos(e4) + 2*a3*m5*x5*cos(e4)*cos(e5) - 4*I6xy*cos(e4)*cos(e5)*cos(e6)^2*sin(e4) - 2*I6zx*cos(e4)^2*cos(e5)*cos(e6)*sin(e5) - a2*m4*y4*cos(e3)*sin(e4) - a2*m5*y5*cos(e5)*sin(e3) - 2*a3*m5*y5*cos(e4)*sin(e5) - 2*a3*m6*y6*cos(e6)*sin(e4) + a2*m5*z5*cos(e3)*sin(e4) - a2*m6*z6*cos(e5)*sin(e3) - 2*a3*m6*z6*cos(e4)*sin(e5) + 2*d4*m6*x6*cos(e6)*sin(e5) + 2*I6yz*cos(e4)^2*cos(e5)*sin(e5)*sin(e6) - a2*m5*x5*sin(e3)*sin(e5) - 2*a3*m6*x6*sin(e4)*sin(e6) - 2*d4*m6*y6*sin(e5)*sin(e6) - 2*I6xy*cos(e4)^2*cos(e5)^2*cos(e6)*sin(e6) + 2*I6yz*cos(e4)*cos(e6)*sin(e4)*sin(e5) + 2*I6zx*cos(e4)*sin(e4)*sin(e5)*sin(e6) - a2*m5*y5*cos(e3)*cos(e4)*sin(e5) - a2*m6*y6*cos(e3)*cos(e6)*sin(e4) - 2*a3*m6*y6*cos(e4)*cos(e5)*sin(e6) - a2*m6*z6*cos(e3)*cos(e4)*sin(e5) - a2*m6*x6*cos(e3)*sin(e4)*sin(e6) - a2*m6*x6*cos(e6)*sin(e3)*sin(e5) + 2*m6*x6*y6*cos(e4)*cos(e5)*sin(e4) + 2*m5*x5*z5*cos(e4)*cos(e5)*sin(e4) + 2*m6*x6*z6*cos(e5)*cos(e6)*sin(e5) + a2*m6*y6*sin(e3)*sin(e5)*sin(e6) - 2*m5*y5*z5*cos(e4)*sin(e4)*sin(e5) - 2*m6*y6*z6*cos(e5)*sin(e5)*sin(e6) - 2*m5*x5*y5*cos(e4)^2*cos(e5)*sin(e5) - 2*m6*x6*y6*cos(e4)^2*cos(e6)*sin(e6) + 2*m6*x6*y6*cos(e5)^2*cos(e6)*sin(e6) + 2*I6xx*cos(e4)*cos(e5)*cos(e6)*sin(e4)*sin(e6) - 2*I6yy*cos(e4)*cos(e5)*cos(e6)*sin(e4)*sin(e6) + a2*m5*x5*cos(e3)*cos(e4)*cos(e5) + 2*a3*m6*x6*cos(e4)*cos(e5)*cos(e6) + 2*m6*y6*z6*cos(e4)*cos(e6)*sin(e4)*sin(e5) + 2*m6*x6*z6*cos(e4)*sin(e4)*sin(e5)*sin(e6) - 4*m6*x6*y6*cos(e4)*cos(e5)*cos(e6)^2*sin(e4) - 2*m6*x6*z6*cos(e4)^2*cos(e5)*cos(e6)*sin(e5) + 2*m6*y6*z6*cos(e4)^2*cos(e5)*sin(e5)*sin(e6) - 2*m6*x6^2*cos(e4)*cos(e5)*cos(e6)*sin(e4)*sin(e6) - 2*m6*x6*y6*cos(e4)^2*cos(e5)^2*cos(e6)*sin(e6) + 2*m6*y6^2*cos(e4)*cos(e5)*cos(e6)*sin(e4)*sin(e6) + a2*m6*x6*cos(e3)*cos(e4)*cos(e5)*cos(e6) - a2*m6*y6*cos(e3)*cos(e4)*cos(e5)*sin(e6),I4xx + I5yy + I3zz + I6zz + a3^2*m4 + a3^2*m5 + a3^2*m6 + d4^2*m4 + d4^2*m5 + d4^2*m6 + m3*x3^2 + m5*x5^2 + m6*x6^2 + m3*y3^2 + m4*y4^2 + m6*y6^2 + m4*z4^2 + m5*z5^2 - I4xx*cos(e4)^2 + I5xx*cos(e5)^2 + I6xx*cos(e4)^2 + I4yy*cos(e4)^2 - I5yy*cos(e4)^2 - I5yy*cos(e5)^2 + I6yy*cos(e5)^2 + I5zz*cos(e4)^2 - I6zz*cos(e4)^2 - I6zz*cos(e5)^2 - I4xy*sin(2*e4) + I5xy*sin(2*e5) + 2*d4*m4*z4 + m4*x4^2*cos(e4)^2 - m5*x5^2*cos(e5)^2 - m6*x6^2*cos(e4)^2 - m4*y4^2*cos(e4)^2 + m5*y5^2*cos(e4)^2 + m5*y5^2*cos(e5)^2 - m6*y6^2*cos(e5)^2 - m5*z5^2*cos(e4)^2 + m6*z6^2*cos(e4)^2 + m6*z6^2*cos(e5)^2 - I5xx*cos(e4)^2*cos(e5)^2 - I6xx*cos(e4)^2*cos(e6)^2 + I6xx*cos(e5)^2*cos(e6)^2 + I5yy*cos(e4)^2*cos(e5)^2 - I6yy*cos(e4)^2*cos(e5)^2 + I6yy*cos(e4)^2*cos(e6)^2 - I6yy*cos(e5)^2*cos(e6)^2 + I6zz*cos(e4)^2*cos(e5)^2 + 2*I6xy*cos(e4)*cos(e5)*sin(e4) + 2*I5zx*cos(e4)*cos(e5)*sin(e4) + 2*I6zx*cos(e5)*cos(e6)*sin(e5) - I6xx*cos(e4)^2*cos(e5)^2*cos(e6)^2 + I6yy*cos(e4)^2*cos(e5)^2*cos(e6)^2 - 2*I5yz*cos(e4)*sin(e4)*sin(e5) - 2*I6yz*cos(e5)*sin(e5)*sin(e6) + 2*a3*m4*x4*cos(e4) - 2*I5xy*cos(e4)^2*cos(e5)*sin(e5) - 2*I6xy*cos(e4)^2*cos(e6)*sin(e6) + 2*I6xy*cos(e5)^2*cos(e6)*sin(e6) + 2*d4*m5*y5*cos(e5) + 2*d4*m6*z6*cos(e5) - 2*a3*m4*y4*sin(e4) + 2*a3*m5*z5*sin(e4) + 2*d4*m5*x5*sin(e5) + m5*x5^2*cos(e4)^2*cos(e5)^2 + m6*x6^2*cos(e4)^2*cos(e6)^2 - m6*x6^2*cos(e5)^2*cos(e6)^2 - m5*y5^2*cos(e4)^2*cos(e5)^2 + m6*y6^2*cos(e4)^2*cos(e5)^2 - m6*y6^2*cos(e4)^2*cos(e6)^2 + m6*y6^2*cos(e5)^2*cos(e6)^2 - m4*x4*y4*sin(2*e4) + m5*x5*y5*sin(2*e5) - m6*z6^2*cos(e4)^2*cos(e5)^2 + m6*x6^2*cos(e4)^2*cos(e5)^2*cos(e6)^2 - m6*y6^2*cos(e4)^2*cos(e5)^2*cos(e6)^2 + 2*a3*m5*x5*cos(e4)*cos(e5) - 4*I6xy*cos(e4)*cos(e5)*cos(e6)^2*sin(e4) - 2*I6zx*cos(e4)^2*cos(e5)*cos(e6)*sin(e5) - 2*a3*m5*y5*cos(e4)*sin(e5) - 2*a3*m6*y6*cos(e6)*sin(e4) - 2*a3*m6*z6*cos(e4)*sin(e5) + 2*d4*m6*x6*cos(e6)*sin(e5) + 2*I6yz*cos(e4)^2*cos(e5)*sin(e5)*sin(e6) - 2*a3*m6*x6*sin(e4)*sin(e6) - 2*d4*m6*y6*sin(e5)*sin(e6) - 2*I6xy*cos(e4)^2*cos(e5)^2*cos(e6)*sin(e6) + 2*I6yz*cos(e4)*cos(e6)*sin(e4)*sin(e5) + 2*I6zx*cos(e4)*sin(e4)*sin(e5)*sin(e6) - 2*a3*m6*y6*cos(e4)*cos(e5)*sin(e6) + 2*m6*x6*y6*cos(e4)*cos(e5)*sin(e4) + 2*m5*x5*z5*cos(e4)*cos(e5)*sin(e4) + 2*m6*x6*z6*cos(e5)*cos(e6)*sin(e5) - 2*m5*y5*z5*cos(e4)*sin(e4)*sin(e5) - 2*m6*y6*z6*cos(e5)*sin(e5)*sin(e6) - 2*m5*x5*y5*cos(e4)^2*cos(e5)*sin(e5) - 2*m6*x6*y6*cos(e4)^2*cos(e6)*sin(e6) + 2*m6*x6*y6*cos(e5)^2*cos(e6)*sin(e6) + 2*I6xx*cos(e4)*cos(e5)*cos(e6)*sin(e4)*sin(e6) - 2*I6yy*cos(e4)*cos(e5)*cos(e6)*sin(e4)*sin(e6) + 2*a3*m6*x6*cos(e4)*cos(e5)*cos(e6) + 2*m6*y6*z6*cos(e4)*cos(e6)*sin(e4)*sin(e5) + 2*m6*x6*z6*cos(e4)*sin(e4)*sin(e5)*sin(e6) - 4*m6*x6*y6*cos(e4)*cos(e5)*cos(e6)^2*sin(e4) - 2*m6*x6*z6*cos(e4)^2*cos(e5)*cos(e6)*sin(e5) + 2*m6*y6*z6*cos(e4)^2*cos(e5)*sin(e5)*sin(e6) - 2*m6*x6^2*cos(e4)*cos(e5)*cos(e6)*sin(e4)*sin(e6) - 2*m6*x6*y6*cos(e4)^2*cos(e5)^2*cos(e6)*sin(e6) + 2*m6*y6^2*cos(e4)*cos(e5)*cos(e6)*sin(e4)*sin(e6),I4yz*cos(e4) - I5xy*sin(e4) + I4zx*sin(e4) - I5yz*cos(e4)*cos(e5) - I6xy*cos(e4)*sin(e5) - I5zx*cos(e4)*sin(e5) - I6zx*cos(e6)*sin(e4) + I6yz*sin(e4)*sin(e6) + 2*I5xy*cos(e5)^2*sin(e4) + I6yz*cos(e4)*cos(e5)*cos(e6) + I6zx*cos(e4)*cos(e5)*sin(e6) - I5xx*cos(e5)*sin(e4)*sin(e5) + I5yy*cos(e5)*sin(e4)*sin(e5) - I6yy*cos(e5)*sin(e4)*sin(e5) + I6zz*cos(e5)*sin(e4)*sin(e5) + 2*I6xy*cos(e4)*cos(e6)^2*sin(e5) + 2*I6zx*cos(e5)^2*cos(e6)*sin(e4) + d4*m4*y4*cos(e4) - d4*m5*z5*cos(e4) + d4*m4*x4*sin(e4) - 2*I6yz*cos(e5)^2*sin(e4)*sin(e6) + m4*y4*z4*cos(e4) - m5*x5*y5*sin(e4) + m4*x4*z4*sin(e4) + m5*x5^2*cos(e5)*sin(e4)*sin(e5) - m5*y5^2*cos(e5)*sin(e4)*sin(e5) + m6*y6^2*cos(e5)*sin(e4)*sin(e5) - m6*z6^2*cos(e5)*sin(e4)*sin(e5) + d4*m6*y6*cos(e4)*cos(e6) + d4*m5*x5*cos(e5)*sin(e4) + d4*m6*x6*cos(e4)*sin(e6) - I6xx*cos(e5)*cos(e6)^2*sin(e4)*sin(e5) + I6yy*cos(e5)*cos(e6)^2*sin(e4)*sin(e5) - m5*y5*z5*cos(e4)*cos(e5) - d4*m5*y5*sin(e4)*sin(e5) - d4*m6*z6*sin(e4)*sin(e5) - m6*x6*y6*cos(e4)*sin(e5) - m5*x5*z5*cos(e4)*sin(e5) - m6*x6*z6*cos(e6)*sin(e4) + m6*y6*z6*sin(e4)*sin(e6) + 2*m5*x5*y5*cos(e5)^2*sin(e4) - I6xx*cos(e4)*cos(e6)*sin(e5)*sin(e6) + I6yy*cos(e4)*cos(e6)*sin(e5)*sin(e6) + d4*m6*x6*cos(e5)*cos(e6)*sin(e4) + m6*y6*z6*cos(e4)*cos(e5)*cos(e6) - d4*m6*y6*cos(e5)*sin(e4)*sin(e6) + m6*x6*z6*cos(e4)*cos(e5)*sin(e6) + m6*x6^2*cos(e5)*cos(e6)^2*sin(e4)*sin(e5) - m6*y6^2*cos(e5)*cos(e6)^2*sin(e4)*sin(e5) + 2*m6*x6*y6*cos(e4)*cos(e6)^2*sin(e5) + 2*m6*x6*z6*cos(e5)^2*cos(e6)*sin(e4) - 2*m6*y6*z6*cos(e5)^2*sin(e4)*sin(e6) - 2*I6xy*cos(e5)*cos(e6)*sin(e4)*sin(e5)*sin(e6) + m6*x6^2*cos(e4)*cos(e6)*sin(e5)*sin(e6) - m6*y6^2*cos(e4)*cos(e6)*sin(e5)*sin(e6) - 2*m6*x6*y6*cos(e5)*cos(e6)*sin(e4)*sin(e5)*sin(e6),I6xx*cos(e4) + I5zz*cos(e4) + I6xy*cos(e5)*sin(e4) + I5zx*cos(e5)*sin(e4) - I5yz*sin(e4)*sin(e5) + m5*x5^2*cos(e4) + m5*y5^2*cos(e4) + m6*y6^2*cos(e4) + m6*z6^2*cos(e4) - I6xx*cos(e4)*cos(e6)^2 + I6yy*cos(e4)*cos(e6)^2 - 2*I6xy*cos(e4)*cos(e6)*sin(e6) + I6yz*cos(e6)*sin(e4)*sin(e5) + I6zx*sin(e4)*sin(e5)*sin(e6) + a3*m5*x5*cos(e5) - 2*I6xy*cos(e5)*cos(e6)^2*sin(e4) - a3*m5*y5*sin(e5) - a3*m6*z6*sin(e5) + m6*x6^2*cos(e4)*cos(e6)^2 - m6*y6^2*cos(e4)*cos(e6)^2 + a3*m6*x6*cos(e5)*cos(e6) + d4*m5*y5*cos(e4)*cos(e5) + d4*m6*z6*cos(e4)*cos(e5) - a3*m6*y6*cos(e5)*sin(e6) + d4*m5*x5*cos(e4)*sin(e5) + m6*x6*y6*cos(e5)*sin(e4) + m5*x5*z5*cos(e5)*sin(e4) - m5*y5*z5*sin(e4)*sin(e5) + I6xx*cos(e5)*cos(e6)*sin(e4)*sin(e6) - I6yy*cos(e5)*cos(e6)*sin(e4)*sin(e6) + d4*m6*x6*cos(e4)*cos(e6)*sin(e5) - d4*m6*y6*cos(e4)*sin(e5)*sin(e6) - 2*m6*x6*y6*cos(e4)*cos(e6)*sin(e6) + m6*y6*z6*cos(e6)*sin(e4)*sin(e5) + m6*x6*z6*sin(e4)*sin(e5)*sin(e6) - 2*m6*x6*y6*cos(e5)*cos(e6)^2*sin(e4) - m6*x6^2*cos(e5)*cos(e6)*sin(e4)*sin(e6) + m6*y6^2*cos(e5)*cos(e6)*sin(e4)*sin(e6),I6yz*cos(e4)*cos(e6) + I6zx*cos(e4)*sin(e6) + I6zz*sin(e4)*sin(e5) + I6zx*cos(e5)*cos(e6)*sin(e4) - I6yz*cos(e5)*sin(e4)*sin(e6) + m6*x6^2*sin(e4)*sin(e5) + m6*y6^2*sin(e4)*sin(e5) - a3*m6*y6*cos(e6)*sin(e5) + d4*m6*x6*cos(e6)*sin(e4) + m6*y6*z6*cos(e4)*cos(e6) - a3*m6*x6*sin(e5)*sin(e6) - d4*m6*y6*sin(e4)*sin(e6) + m6*x6*z6*cos(e4)*sin(e6) + d4*m6*y6*cos(e4)*cos(e5)*cos(e6) + d4*m6*x6*cos(e4)*cos(e5)*sin(e6) + m6*x6*z6*cos(e5)*cos(e6)*sin(e4) - m6*y6*z6*cos(e5)*sin(e4)*sin(e6);
 I4yz*(cos(e2)*cos(e3)*sin(e4) - sin(e2)*sin(e3)*sin(e4)) - I4zz*sin(e2 + e3) - (I6xx*cos(e6)*sin(e5) - I6zx*cos(e5) + I6xy*sin(e5)*sin(e6))*(cos(e2)*cos(e3)*sin(e4)*sin(e6) + cos(e2)*cos(e6)*sin(e3)*sin(e5) + cos(e3)*cos(e6)*sin(e2)*sin(e5) - sin(e2)*sin(e3)*sin(e4)*sin(e6) - cos(e2)*cos(e3)*cos(e4)*cos(e5)*cos(e6) + cos(e4)*cos(e5)*cos(e6)*sin(e2)*sin(e3)) - I4zx*(cos(e2)*cos(e3)*cos(e4) - cos(e4)*sin(e2)*sin(e3)) - (I6yz*cos(e5) + I6xy*cos(e6)*sin(e5) + I6yy*sin(e5)*sin(e6))*(cos(e6)*sin(e2)*sin(e3)*sin(e4) - cos(e2)*cos(e3)*cos(e6)*sin(e4) + cos(e2)*sin(e3)*sin(e5)*sin(e6) + cos(e3)*sin(e2)*sin(e5)*sin(e6) - cos(e2)*cos(e3)*cos(e4)*cos(e5)*sin(e6) + cos(e4)*cos(e5)*sin(e2)*sin(e3)*sin(e6)) - (I6zz*cos(e5) - I6zx*cos(e6)*sin(e5) + I6yz*sin(e5)*sin(e6))*(cos(e2)*cos(e5)*sin(e3) + cos(e3)*cos(e5)*sin(e2) + cos(e2)*cos(e3)*cos(e4)*sin(e5) - cos(e4)*sin(e2)*sin(e3)*sin(e5)) - (cos(e2)*cos(e3)*sin(e4) - sin(e2)*sin(e3)*sin(e4))*(I5yz*cos(e5) + I5zx*sin(e5)) + (I5xy*cos(e5) - I5xx*sin(e5))*(cos(e2)*sin(e3)*sin(e5) + cos(e3)*sin(e2)*sin(e5) - cos(e2)*cos(e3)*cos(e4)*cos(e5) + cos(e4)*cos(e5)*sin(e2)*sin(e3)) - (I5yy*cos(e5) - I5xy*sin(e5))*(cos(e2)*cos(e5)*sin(e3) + cos(e3)*cos(e5)*sin(e2) + cos(e2)*cos(e3)*cos(e4)*sin(e5) - cos(e4)*sin(e2)*sin(e3)*sin(e5)) - m4*(x4*(cos(e1)*cos(e4) + sin(e2 + e3)*sin(e1)*sin(e4)) - y4*(cos(e1)*sin(e4) - sin(e2 + e3)*cos(e4)*sin(e1)))*(cos(e1)*(a1 + d4*cos(e2 + e3) + a3*sin(e2 + e3) + a2*sin(e2)) + x4*(sin(e1)*sin(e4) + sin(e2 + e3)*cos(e1)*cos(e4)) + y4*(cos(e4)*sin(e1) - sin(e2 + e3)*cos(e1)*sin(e4)) + z4*cos(e2 + e3)*cos(e1)) + m6*(x6*(sin(e6)*(cos(e1)*sin(e4) - sin(e2 + e3)*cos(e4)*sin(e1)) - cos(e5)*cos(e6)*(cos(e1)*cos(e4) + sin(e2 + e3)*sin(e1)*sin(e4))) + y6*(cos(e6)*(cos(e1)*sin(e4) - sin(e2 + e3)*cos(e4)*sin(e1)) + cos(e5)*sin(e6)*(cos(e1)*cos(e4) + sin(e2 + e3)*sin(e1)*sin(e4))) + z6*sin(e5)*(cos(e1)*cos(e4) + sin(e2 + e3)*sin(e1)*sin(e4)))*(cos(e1)*(a1 + d4*cos(e2 + e3) + a3*sin(e2 + e3) + a2*sin(e2)) + x6*(sin(e6)*(cos(e4)*sin(e1) - sin(e2 + e3)*cos(e1)*sin(e4)) + cos(e6)*(cos(e5)*(sin(e1)*sin(e4) + sin(e2 + e3)*cos(e1)*cos(e4)) + cos(e2 + e3)*cos(e1)*sin(e5))) + y6*(cos(e6)*(cos(e4)*sin(e1) - sin(e2 + e3)*cos(e1)*sin(e4)) - sin(e6)*(cos(e5)*(sin(e1)*sin(e4) + sin(e2 + e3)*cos(e1)*cos(e4)) + cos(e2 + e3)*cos(e1)*sin(e5))) - z6*(sin(e5)*(sin(e1)*sin(e4) + sin(e2 + e3)*cos(e1)*cos(e4)) - cos(e2 + e3)*cos(e1)*cos(e5))) - m4*(x4*(cos(e4)*sin(e1) - sin(e2 + e3)*cos(e1)*sin(e4)) - y4*(sin(e1)*sin(e4) + sin(e2 + e3)*cos(e1)*cos(e4)))*(sin(e1)*(a1 + d4*cos(e2 + e3) + a3*sin(e2 + e3) + a2*sin(e2)) - x4*(cos(e1)*sin(e4) - sin(e2 + e3)*cos(e4)*sin(e1)) - y4*(cos(e1)*cos(e4) + sin(e2 + e3)*sin(e1)*sin(e4)) + z4*cos(e2 + e3)*sin(e1)) - m5*(z5*(cos(e1)*sin(e4) - sin(e2 + e3)*cos(e4)*sin(e1)) + x5*cos(e5)*(cos(e1)*cos(e4) + sin(e2 + e3)*sin(e1)*sin(e4)) - y5*sin(e5)*(cos(e1)*cos(e4) + sin(e2 + e3)*sin(e1)*sin(e4)))*(cos(e1)*(a1 + d4*cos(e2 + e3) + a3*sin(e2 + e3) + a2*sin(e2)) - z5*(cos(e4)*sin(e1) - sin(e2 + e3)*cos(e1)*sin(e4)) + x5*(cos(e5)*(sin(e1)*sin(e4) + sin(e2 + e3)*cos(e1)*cos(e4)) + cos(e2 + e3)*cos(e1)*sin(e5)) - y5*(sin(e5)*(sin(e1)*sin(e4) + sin(e2 + e3)*cos(e1)*cos(e4)) - cos(e2 + e3)*cos(e1)*cos(e5))) + m6*(x6*(sin(e6)*(sin(e1)*sin(e4) + sin(e2 + e3)*cos(e1)*cos(e4)) - cos(e5)*cos(e6)*(cos(e4)*sin(e1) - sin(e2 + e3)*cos(e1)*sin(e4))) + y6*(cos(e6)*(sin(e1)*sin(e4) + sin(e2 + e3)*cos(e1)*cos(e4)) + cos(e5)*sin(e6)*(cos(e4)*sin(e1) - sin(e2 + e3)*cos(e1)*sin(e4))) + z6*sin(e5)*(cos(e4)*sin(e1) - sin(e2 + e3)*cos(e1)*sin(e4)))*(sin(e1)*(a1 + d4*cos(e2 + e3) + a3*sin(e2 + e3) + a2*sin(e2)) - x6*(sin(e6)*(cos(e1)*cos(e4) + sin(e2 + e3)*sin(e1)*sin(e4)) + cos(e6)*(cos(e5)*(cos(e1)*sin(e4) - sin(e2 + e3)*cos(e4)*sin(e1)) - cos(e2 + e3)*sin(e1)*sin(e5))) - y6*(cos(e6)*(cos(e1)*cos(e4) + sin(e2 + e3)*sin(e1)*sin(e4)) - sin(e6)*(cos(e5)*(cos(e1)*sin(e4) - sin(e2 + e3)*cos(e4)*sin(e1)) - cos(e2 + e3)*sin(e1)*sin(e5))) + z6*(sin(e5)*(cos(e1)*sin(e4) - sin(e2 + e3)*cos(e4)*sin(e1)) + cos(e2 + e3)*cos(e5)*sin(e1))) - m5*(z5*(sin(e1)*sin(e4) + sin(e2 + e3)*cos(e1)*cos(e4)) + x5*cos(e5)*(cos(e4)*sin(e1) - sin(e2 + e3)*cos(e1)*sin(e4)) - y5*sin(e5)*(cos(e4)*sin(e1) - sin(e2 + e3)*cos(e1)*sin(e4)))*(sin(e1)*(a1 + d4*cos(e2 + e3) + a3*sin(e2 + e3) + a2*sin(e2)) + z5*(cos(e1)*cos(e4) + sin(e2 + e3)*sin(e1)*sin(e4)) - x5*(cos(e5)*(cos(e1)*sin(e4) - sin(e2 + e3)*cos(e4)*sin(e1)) - cos(e2 + e3)*sin(e1)*sin(e5)) + y5*(sin(e5)*(cos(e1)*sin(e4) - sin(e2 + e3)*cos(e4)*sin(e1)) + cos(e2 + e3)*cos(e5)*sin(e1))),I4yz*cos(e4) - I5xy*sin(e4) + I4zx*sin(e4) - I5yz*cos(e4)*cos(e5) - I6xy*cos(e4)*sin(e5) - I5zx*cos(e4)*sin(e5) - I6zx*cos(e6)*sin(e4) + I6yz*sin(e4)*sin(e6) + 2*I5xy*cos(e5)^2*sin(e4) + I6yz*cos(e4)*cos(e5)*cos(e6) + I6zx*cos(e4)*cos(e5)*sin(e6) - I5xx*cos(e5)*sin(e4)*sin(e5) + I5yy*cos(e5)*sin(e4)*sin(e5) - I6yy*cos(e5)*sin(e4)*sin(e5) + I6zz*cos(e5)*sin(e4)*sin(e5) + 2*I6xy*cos(e4)*cos(e6)^2*sin(e5) + 2*I6zx*cos(e5)^2*cos(e6)*sin(e4) + d4*m4*y4*cos(e4) - d4*m5*z5*cos(e4) + d4*m4*x4*sin(e4) - 2*I6yz*cos(e5)^2*sin(e4)*sin(e6) + m4*y4*z4*cos(e4) - m5*x5*y5*sin(e4) + m4*x4*z4*sin(e4) + m5*x5^2*cos(e5)*sin(e4)*sin(e5) - m5*y5^2*cos(e5)*sin(e4)*sin(e5) + m6*y6^2*cos(e5)*sin(e4)*sin(e5) - m6*z6^2*cos(e5)*sin(e4)*sin(e5) + d4*m6*y6*cos(e4)*cos(e6) - a2*m4*y4*cos(e4)*sin(e3) + a2*m5*z5*cos(e4)*sin(e3) + d4*m5*x5*cos(e5)*sin(e4) + d4*m6*x6*cos(e4)*sin(e6) - I6xx*cos(e5)*cos(e6)^2*sin(e4)*sin(e5) + I6yy*cos(e5)*cos(e6)^2*sin(e4)*sin(e5) - m5*y5*z5*cos(e4)*cos(e5) - a2*m4*x4*sin(e3)*sin(e4) - d4*m5*y5*sin(e4)*sin(e5) - d4*m6*z6*sin(e4)*sin(e5) - m6*x6*y6*cos(e4)*sin(e5) - m5*x5*z5*cos(e4)*sin(e5) - m6*x6*z6*cos(e6)*sin(e4) + m6*y6*z6*sin(e4)*sin(e6) + 2*m5*x5*y5*cos(e5)^2*sin(e4) - I6xx*cos(e4)*cos(e6)*sin(e5)*sin(e6) + I6yy*cos(e4)*cos(e6)*sin(e5)*sin(e6) - a2*m6*y6*cos(e4)*cos(e6)*sin(e3) + d4*m6*x6*cos(e5)*cos(e6)*sin(e4) + m6*y6*z6*cos(e4)*cos(e5)*cos(e6) - a2*m5*x5*cos(e5)*sin(e3)*sin(e4) - a2*m6*x6*cos(e4)*sin(e3)*sin(e6) - d4*m6*y6*cos(e5)*sin(e4)*sin(e6) + m6*x6*z6*cos(e4)*cos(e5)*sin(e6) + a2*m5*y5*sin(e3)*sin(e4)*sin(e5) + a2*m6*z6*sin(e3)*sin(e4)*sin(e5) + m6*x6^2*cos(e5)*cos(e6)^2*sin(e4)*sin(e5) - m6*y6^2*cos(e5)*cos(e6)^2*sin(e4)*sin(e5) + 2*m6*x6*y6*cos(e4)*cos(e6)^2*sin(e5) + 2*m6*x6*z6*cos(e5)^2*cos(e6)*sin(e4) - 2*m6*y6*z6*cos(e5)^2*sin(e4)*sin(e6) - 2*I6xy*cos(e5)*cos(e6)*sin(e4)*sin(e5)*sin(e6) + m6*x6^2*cos(e4)*cos(e6)*sin(e5)*sin(e6) - m6*y6^2*cos(e4)*cos(e6)*sin(e5)*sin(e6) - a2*m6*x6*cos(e5)*cos(e6)*sin(e3)*sin(e4) + a2*m6*y6*cos(e5)*sin(e3)*sin(e4)*sin(e6) - 2*m6*x6*y6*cos(e5)*cos(e6)*sin(e4)*sin(e5)*sin(e6),I4yz*cos(e4) - I5xy*sin(e4) + I4zx*sin(e4) - I5yz*cos(e4)*cos(e5) - I6xy*cos(e4)*sin(e5) - I5zx*cos(e4)*sin(e5) - I6zx*cos(e6)*sin(e4) + I6yz*sin(e4)*sin(e6) + 2*I5xy*cos(e5)^2*sin(e4) + I6yz*cos(e4)*cos(e5)*cos(e6) + I6zx*cos(e4)*cos(e5)*sin(e6) - I5xx*cos(e5)*sin(e4)*sin(e5) + I5yy*cos(e5)*sin(e4)*sin(e5) - I6yy*cos(e5)*sin(e4)*sin(e5) + I6zz*cos(e5)*sin(e4)*sin(e5) + 2*I6xy*cos(e4)*cos(e6)^2*sin(e5) + 2*I6zx*cos(e5)^2*cos(e6)*sin(e4) + d4*m4*y4*cos(e4) - d4*m5*z5*cos(e4) + d4*m4*x4*sin(e4) - 2*I6yz*cos(e5)^2*sin(e4)*sin(e6) + m4*y4*z4*cos(e4) - m5*x5*y5*sin(e4) + m4*x4*z4*sin(e4) + m5*x5^2*cos(e5)*sin(e4)*sin(e5) - m5*y5^2*cos(e5)*sin(e4)*sin(e5) + m6*y6^2*cos(e5)*sin(e4)*sin(e5) - m6*z6^2*cos(e5)*sin(e4)*sin(e5) + d4*m6*y6*cos(e4)*cos(e6) + d4*m5*x5*cos(e5)*sin(e4) + d4*m6*x6*cos(e4)*sin(e6) - I6xx*cos(e5)*cos(e6)^2*sin(e4)*sin(e5) + I6yy*cos(e5)*cos(e6)^2*sin(e4)*sin(e5) - m5*y5*z5*cos(e4)*cos(e5) - d4*m5*y5*sin(e4)*sin(e5) - d4*m6*z6*sin(e4)*sin(e5) - m6*x6*y6*cos(e4)*sin(e5) - m5*x5*z5*cos(e4)*sin(e5) - m6*x6*z6*cos(e6)*sin(e4) + m6*y6*z6*sin(e4)*sin(e6) + 2*m5*x5*y5*cos(e5)^2*sin(e4) - I6xx*cos(e4)*cos(e6)*sin(e5)*sin(e6) + I6yy*cos(e4)*cos(e6)*sin(e5)*sin(e6) + d4*m6*x6*cos(e5)*cos(e6)*sin(e4) + m6*y6*z6*cos(e4)*cos(e5)*cos(e6) - d4*m6*y6*cos(e5)*sin(e4)*sin(e6) + m6*x6*z6*cos(e4)*cos(e5)*sin(e6) + m6*x6^2*cos(e5)*cos(e6)^2*sin(e4)*sin(e5) - m6*y6^2*cos(e5)*cos(e6)^2*sin(e4)*sin(e5) + 2*m6*x6*y6*cos(e4)*cos(e6)^2*sin(e5) + 2*m6*x6*z6*cos(e5)^2*cos(e6)*sin(e4) - 2*m6*y6*z6*cos(e5)^2*sin(e4)*sin(e6) - 2*I6xy*cos(e5)*cos(e6)*sin(e4)*sin(e5)*sin(e6) + m6*x6^2*cos(e4)*cos(e6)*sin(e5)*sin(e6) - m6*y6^2*cos(e4)*cos(e6)*sin(e5)*sin(e6) - 2*m6*x6*y6*cos(e5)*cos(e6)*sin(e4)*sin(e5)*sin(e6),I5xx + I6yy + I4zz + m4*x4^2 + m6*x6^2 + m4*y4^2 + m5*y5^2 + m5*z5^2 + m6*z6^2 - I5xx*cos(e5)^2 + I6xx*cos(e6)^2 + I5yy*cos(e5)^2 - I6yy*cos(e5)^2 - I6yy*cos(e6)^2 + I6zz*cos(e5)^2 - I5xy*sin(2*e5) + I6xy*sin(2*e6) + m5*x5^2*cos(e5)^2 - m6*x6^2*cos(e6)^2 - m5*y5^2*cos(e5)^2 + m6*y6^2*cos(e5)^2 + m6*y6^2*cos(e6)^2 - m6*z6^2*cos(e5)^2 - I6xx*cos(e5)^2*cos(e6)^2 + I6yy*cos(e5)^2*cos(e6)^2 - 2*I6zx*cos(e5)*cos(e6)*sin(e5) + 2*I6yz*cos(e5)*sin(e5)*sin(e6) - 2*I6xy*cos(e5)^2*cos(e6)*sin(e6) + m6*x6^2*cos(e5)^2*cos(e6)^2 - m6*y6^2*cos(e5)^2*cos(e6)^2 - m5*x5*y5*sin(2*e5) + m6*x6*y6*sin(2*e6) - 2*m6*x6*z6*cos(e5)*cos(e6)*sin(e5) + 2*m6*y6*z6*cos(e5)*sin(e5)*sin(e6) - 2*m6*x6*y6*cos(e5)^2*cos(e6)*sin(e6),I6yz*cos(e5)*cos(e6) - I6xy*sin(e5) - I5zx*sin(e5) - I5yz*cos(e5) + I6zx*cos(e5)*sin(e6) + 2*I6xy*cos(e6)^2*sin(e5) - I6xx*cos(e6)*sin(e5)*sin(e6) + I6yy*cos(e6)*sin(e5)*sin(e6) - m5*y5*z5*cos(e5) - m6*x6*y6*sin(e5) - m5*x5*z5*sin(e5) + m6*x6^2*cos(e6)*sin(e5)*sin(e6) - m6*y6^2*cos(e6)*sin(e5)*sin(e6) + m6*y6*z6*cos(e5)*cos(e6) + m6*x6*z6*cos(e5)*sin(e6) + 2*m6*x6*y6*cos(e6)^2*sin(e5),I6zz*cos(e5) - I6zx*cos(e6)*sin(e5) + I6yz*sin(e5)*sin(e6) + m6*x6^2*cos(e5) + m6*y6^2*cos(e5) - m6*x6*z6*cos(e6)*sin(e5) + m6*y6*z6*sin(e5)*sin(e6);
 I5zz*(cos(e2)*cos(e3)*sin(e4) - sin(e2)*sin(e3)*sin(e4)) - (I6yy*cos(e6) - I6xy*sin(e6))*(cos(e6)*sin(e2)*sin(e3)*sin(e4) - cos(e2)*cos(e3)*cos(e6)*sin(e4) + cos(e2)*sin(e3)*sin(e5)*sin(e6) + cos(e3)*sin(e2)*sin(e5)*sin(e6) - cos(e2)*cos(e3)*cos(e4)*cos(e5)*sin(e6) + cos(e4)*cos(e5)*sin(e2)*sin(e3)*sin(e6)) - (I6xy*cos(e6) - I6xx*sin(e6))*(cos(e2)*cos(e3)*sin(e4)*sin(e6) + cos(e2)*cos(e6)*sin(e3)*sin(e5) + cos(e3)*cos(e6)*sin(e2)*sin(e5) - sin(e2)*sin(e3)*sin(e4)*sin(e6) - cos(e2)*cos(e3)*cos(e4)*cos(e5)*cos(e6) + cos(e4)*cos(e5)*cos(e6)*sin(e2)*sin(e3)) + I5yz*(cos(e2)*cos(e5)*sin(e3) + cos(e3)*cos(e5)*sin(e2) + cos(e2)*cos(e3)*cos(e4)*sin(e5) - cos(e4)*sin(e2)*sin(e3)*sin(e5)) + I5zx*(cos(e2)*sin(e3)*sin(e5) + cos(e3)*sin(e2)*sin(e5) - cos(e2)*cos(e3)*cos(e4)*cos(e5) + cos(e4)*cos(e5)*sin(e2)*sin(e3)) - (I6yz*cos(e6) + I6zx*sin(e6))*(cos(e2)*cos(e5)*sin(e3) + cos(e3)*cos(e5)*sin(e2) + cos(e2)*cos(e3)*cos(e4)*sin(e5) - cos(e4)*sin(e2)*sin(e3)*sin(e5)) + m5*(x5*(sin(e5)*(cos(e1)*sin(e4) - sin(e2 + e3)*cos(e4)*sin(e1)) + cos(e2 + e3)*cos(e5)*sin(e1)) + y5*(cos(e5)*(cos(e1)*sin(e4) - sin(e2 + e3)*cos(e4)*sin(e1)) - cos(e2 + e3)*sin(e1)*sin(e5)))*(cos(e1)*(a1 + d4*cos(e2 + e3) + a3*sin(e2 + e3) + a2*sin(e2)) - z5*(cos(e4)*sin(e1) - sin(e2 + e3)*cos(e1)*sin(e4)) + x5*(cos(e5)*(sin(e1)*sin(e4) + sin(e2 + e3)*cos(e1)*cos(e4)) + cos(e2 + e3)*cos(e1)*sin(e5)) - y5*(sin(e5)*(sin(e1)*sin(e4) + sin(e2 + e3)*cos(e1)*cos(e4)) - cos(e2 + e3)*cos(e1)*cos(e5))) + m5*(x5*(sin(e5)*(sin(e1)*sin(e4) + sin(e2 + e3)*cos(e1)*cos(e4)) - cos(e2 + e3)*cos(e1)*cos(e5)) + y5*(cos(e5)*(sin(e1)*sin(e4) + sin(e2 + e3)*cos(e1)*cos(e4)) + cos(e2 + e3)*cos(e1)*sin(e5)))*(sin(e1)*(a1 + d4*cos(e2 + e3) + a3*sin(e2 + e3) + a2*sin(e2)) + z5*(cos(e1)*cos(e4) + sin(e2 + e3)*sin(e1)*sin(e4)) - x5*(cos(e5)*(cos(e1)*sin(e4) - sin(e2 + e3)*cos(e4)*sin(e1)) - cos(e2 + e3)*sin(e1)*sin(e5)) + y5*(sin(e5)*(cos(e1)*sin(e4) - sin(e2 + e3)*cos(e4)*sin(e1)) + cos(e2 + e3)*cos(e5)*sin(e1))) + m6*(z6*(cos(e5)*(cos(e1)*sin(e4) - sin(e2 + e3)*cos(e4)*sin(e1)) - cos(e2 + e3)*sin(e1)*sin(e5)) + x6*cos(e6)*(sin(e5)*(cos(e1)*sin(e4) - sin(e2 + e3)*cos(e4)*sin(e1)) + cos(e2 + e3)*cos(e5)*sin(e1)) - y6*sin(e6)*(sin(e5)*(cos(e1)*sin(e4) - sin(e2 + e3)*cos(e4)*sin(e1)) + cos(e2 + e3)*cos(e5)*sin(e1)))*(cos(e1)*(a1 + d4*cos(e2 + e3) + a3*sin(e2 + e3) + a2*sin(e2)) + x6*(sin(e6)*(cos(e4)*sin(e1) - sin(e2 + e3)*cos(e1)*sin(e4)) + cos(e6)*(cos(e5)*(sin(e1)*sin(e4) + sin(e2 + e3)*cos(e1)*cos(e4)) + cos(e2 + e3)*cos(e1)*sin(e5))) + y6*(cos(e6)*(cos(e4)*sin(e1) - sin(e2 + e3)*cos(e1)*sin(e4)) - sin(e6)*(cos(e5)*(sin(e1)*sin(e4) + sin(e2 + e3)*cos(e1)*cos(e4)) + cos(e2 + e3)*cos(e1)*sin(e5))) - z6*(sin(e5)*(sin(e1)*sin(e4) + sin(e2 + e3)*cos(e1)*cos(e4)) - cos(e2 + e3)*cos(e1)*cos(e5))) + m6*(z6*(cos(e5)*(sin(e1)*sin(e4) + sin(e2 + e3)*cos(e1)*cos(e4)) + cos(e2 + e3)*cos(e1)*sin(e5)) + x6*cos(e6)*(sin(e5)*(sin(e1)*sin(e4) + sin(e2 + e3)*cos(e1)*cos(e4)) - cos(e2 + e3)*cos(e1)*cos(e5)) - y6*sin(e6)*(sin(e5)*(sin(e1)*sin(e4) + sin(e2 + e3)*cos(e1)*cos(e4)) - cos(e2 + e3)*cos(e1)*cos(e5)))*(sin(e1)*(a1 + d4*cos(e2 + e3) + a3*sin(e2 + e3) + a2*sin(e2)) - x6*(sin(e6)*(cos(e1)*cos(e4) + sin(e2 + e3)*sin(e1)*sin(e4)) + cos(e6)*(cos(e5)*(cos(e1)*sin(e4) - sin(e2 + e3)*cos(e4)*sin(e1)) - cos(e2 + e3)*sin(e1)*sin(e5))) - y6*(cos(e6)*(cos(e1)*cos(e4) + sin(e2 + e3)*sin(e1)*sin(e4)) - sin(e6)*(cos(e5)*(cos(e1)*sin(e4) - sin(e2 + e3)*cos(e4)*sin(e1)) - cos(e2 + e3)*sin(e1)*sin(e5))) + z6*(sin(e5)*(cos(e1)*sin(e4) - sin(e2 + e3)*cos(e4)*sin(e1)) + cos(e2 + e3)*cos(e5)*sin(e1))),I6xx*cos(e4) + I5zz*cos(e4) + I6xy*cos(e5)*sin(e4) + I5zx*cos(e5)*sin(e4) - I5yz*sin(e4)*sin(e5) + m5*x5^2*cos(e4) + m5*y5^2*cos(e4) + m6*y6^2*cos(e4) + m6*z6^2*cos(e4) - I6xx*cos(e4)*cos(e6)^2 + I6yy*cos(e4)*cos(e6)^2 - 2*I6xy*cos(e4)*cos(e6)*sin(e6) + I6yz*cos(e6)*sin(e4)*sin(e5) + I6zx*sin(e4)*sin(e5)*sin(e6) + a3*m5*x5*cos(e5) - 2*I6xy*cos(e5)*cos(e6)^2*sin(e4) - a3*m5*y5*sin(e5) - a3*m6*z6*sin(e5) + m6*x6^2*cos(e4)*cos(e6)^2 - m6*y6^2*cos(e4)*cos(e6)^2 + a2*m5*x5*cos(e3)*cos(e5) + a3*m6*x6*cos(e5)*cos(e6) + d4*m5*y5*cos(e4)*cos(e5) + d4*m6*z6*cos(e4)*cos(e5) - a2*m5*y5*cos(e3)*sin(e5) - a3*m6*y6*cos(e5)*sin(e6) - a2*m6*z6*cos(e3)*sin(e5) + d4*m5*x5*cos(e4)*sin(e5) + m6*x6*y6*cos(e5)*sin(e4) + m5*x5*z5*cos(e5)*sin(e4) - m5*y5*z5*sin(e4)*sin(e5) + I6xx*cos(e5)*cos(e6)*sin(e4)*sin(e6) - I6yy*cos(e5)*cos(e6)*sin(e4)*sin(e6) - a2*m5*y5*cos(e4)*cos(e5)*sin(e3) - a2*m6*y6*cos(e3)*cos(e5)*sin(e6) - a2*m6*z6*cos(e4)*cos(e5)*sin(e3) + d4*m6*x6*cos(e4)*cos(e6)*sin(e5) - a2*m5*x5*cos(e4)*sin(e3)*sin(e5) - d4*m6*y6*cos(e4)*sin(e5)*sin(e6) - 2*m6*x6*y6*cos(e4)*cos(e6)*sin(e6) + m6*y6*z6*cos(e6)*sin(e4)*sin(e5) + m6*x6*z6*sin(e4)*sin(e5)*sin(e6) - 2*m6*x6*y6*cos(e5)*cos(e6)^2*sin(e4) - m6*x6^2*cos(e5)*cos(e6)*sin(e4)*sin(e6) + m6*y6^2*cos(e5)*cos(e6)*sin(e4)*sin(e6) + a2*m6*x6*cos(e3)*cos(e5)*cos(e6) - a2*m6*x6*cos(e4)*cos(e6)*sin(e3)*sin(e5) + a2*m6*y6*cos(e4)*sin(e3)*sin(e5)*sin(e6),I6xx*cos(e4) + I5zz*cos(e4) + I6xy*cos(e5)*sin(e4) + I5zx*cos(e5)*sin(e4) - I5yz*sin(e4)*sin(e5) + m5*x5^2*cos(e4) + m5*y5^2*cos(e4) + m6*y6^2*cos(e4) + m6*z6^2*cos(e4) - I6xx*cos(e4)*cos(e6)^2 + I6yy*cos(e4)*cos(e6)^2 - 2*I6xy*cos(e4)*cos(e6)*sin(e6) + I6yz*cos(e6)*sin(e4)*sin(e5) + I6zx*sin(e4)*sin(e5)*sin(e6) + a3*m5*x5*cos(e5) - 2*I6xy*cos(e5)*cos(e6)^2*sin(e4) - a3*m5*y5*sin(e5) - a3*m6*z6*sin(e5) + m6*x6^2*cos(e4)*cos(e6)^2 - m6*y6^2*cos(e4)*cos(e6)^2 + a3*m6*x6*cos(e5)*cos(e6) + d4*m5*y5*cos(e4)*cos(e5) + d4*m6*z6*cos(e4)*cos(e5) - a3*m6*y6*cos(e5)*sin(e6) + d4*m5*x5*cos(e4)*sin(e5) + m6*x6*y6*cos(e5)*sin(e4) + m5*x5*z5*cos(e5)*sin(e4) - m5*y5*z5*sin(e4)*sin(e5) + I6xx*cos(e5)*cos(e6)*sin(e4)*sin(e6) - I6yy*cos(e5)*cos(e6)*sin(e4)*sin(e6) + d4*m6*x6*cos(e4)*cos(e6)*sin(e5) - d4*m6*y6*cos(e4)*sin(e5)*sin(e6) - 2*m6*x6*y6*cos(e4)*cos(e6)*sin(e6) + m6*y6*z6*cos(e6)*sin(e4)*sin(e5) + m6*x6*z6*sin(e4)*sin(e5)*sin(e6) - 2*m6*x6*y6*cos(e5)*cos(e6)^2*sin(e4) - m6*x6^2*cos(e5)*cos(e6)*sin(e4)*sin(e6) + m6*y6^2*cos(e5)*cos(e6)*sin(e4)*sin(e6),I6yz*cos(e5)*cos(e6) - I6xy*sin(e5) - I5zx*sin(e5) - I5yz*cos(e5) + I6zx*cos(e5)*sin(e6) + 2*I6xy*cos(e6)^2*sin(e5) - I6xx*cos(e6)*sin(e5)*sin(e6) + I6yy*cos(e6)*sin(e5)*sin(e6) - m5*y5*z5*cos(e5) - m6*x6*y6*sin(e5) - m5*x5*z5*sin(e5) + m6*x6^2*cos(e6)*sin(e5)*sin(e6) - m6*y6^2*cos(e6)*sin(e5)*sin(e6) + m6*y6*z6*cos(e5)*cos(e6) + m6*x6*z6*cos(e5)*sin(e6) + 2*m6*x6*y6*cos(e6)^2*sin(e5),I6xx + I5zz + m5*x5^2 + m5*y5^2 + m6*y6^2 + m6*z6^2 - I6xx*cos(e6)^2 + I6yy*cos(e6)^2 - I6xy*sin(2*e6) + m6*x6^2*cos(e6)^2 - m6*y6^2*cos(e6)^2 - m6*x6*y6*sin(2*e6),I6yz*cos(e6) + I6zx*sin(e6) + m6*y6*z6*cos(e6) + m6*x6*z6*sin(e6);
 I6zx*(cos(e2)*cos(e3)*sin(e4)*sin(e6) + cos(e2)*cos(e6)*sin(e3)*sin(e5) + cos(e3)*cos(e6)*sin(e2)*sin(e5) - sin(e2)*sin(e3)*sin(e4)*sin(e6) - cos(e2)*cos(e3)*cos(e4)*cos(e5)*cos(e6) + cos(e4)*cos(e5)*cos(e6)*sin(e2)*sin(e3)) - I6yz*(cos(e6)*sin(e2)*sin(e3)*sin(e4) - cos(e2)*cos(e3)*cos(e6)*sin(e4) + cos(e2)*sin(e3)*sin(e5)*sin(e6) + cos(e3)*sin(e2)*sin(e5)*sin(e6) - cos(e2)*cos(e3)*cos(e4)*cos(e5)*sin(e6) + cos(e4)*cos(e5)*sin(e2)*sin(e3)*sin(e6)) - I6zz*(cos(e2)*cos(e5)*sin(e3) + cos(e3)*cos(e5)*sin(e2) + cos(e2)*cos(e3)*cos(e4)*sin(e5) - cos(e4)*sin(e2)*sin(e3)*sin(e5)) - m6*(x6*(cos(e6)*(cos(e1)*cos(e4) + sin(e2 + e3)*sin(e1)*sin(e4)) - sin(e6)*(cos(e5)*(cos(e1)*sin(e4) - sin(e2 + e3)*cos(e4)*sin(e1)) - cos(e2 + e3)*sin(e1)*sin(e5))) - y6*(sin(e6)*(cos(e1)*cos(e4) + sin(e2 + e3)*sin(e1)*sin(e4)) + cos(e6)*(cos(e5)*(cos(e1)*sin(e4) - sin(e2 + e3)*cos(e4)*sin(e1)) - cos(e2 + e3)*sin(e1)*sin(e5))))*(cos(e1)*(a1 + d4*cos(e2 + e3) + a3*sin(e2 + e3) + a2*sin(e2)) + x6*(sin(e6)*(cos(e4)*sin(e1) - sin(e2 + e3)*cos(e1)*sin(e4)) + cos(e6)*(cos(e5)*(sin(e1)*sin(e4) + sin(e2 + e3)*cos(e1)*cos(e4)) + cos(e2 + e3)*cos(e1)*sin(e5))) + y6*(cos(e6)*(cos(e4)*sin(e1) - sin(e2 + e3)*cos(e1)*sin(e4)) - sin(e6)*(cos(e5)*(sin(e1)*sin(e4) + sin(e2 + e3)*cos(e1)*cos(e4)) + cos(e2 + e3)*cos(e1)*sin(e5))) - z6*(sin(e5)*(sin(e1)*sin(e4) + sin(e2 + e3)*cos(e1)*cos(e4)) - cos(e2 + e3)*cos(e1)*cos(e5))) - m6*(x6*(cos(e6)*(cos(e4)*sin(e1) - sin(e2 + e3)*cos(e1)*sin(e4)) - sin(e6)*(cos(e5)*(sin(e1)*sin(e4) + sin(e2 + e3)*cos(e1)*cos(e4)) + cos(e2 + e3)*cos(e1)*sin(e5))) - y6*(sin(e6)*(cos(e4)*sin(e1) - sin(e2 + e3)*cos(e1)*sin(e4)) + cos(e6)*(cos(e5)*(sin(e1)*sin(e4) + sin(e2 + e3)*cos(e1)*cos(e4)) + cos(e2 + e3)*cos(e1)*sin(e5))))*(sin(e1)*(a1 + d4*cos(e2 + e3) + a3*sin(e2 + e3) + a2*sin(e2)) - x6*(sin(e6)*(cos(e1)*cos(e4) + sin(e2 + e3)*sin(e1)*sin(e4)) + cos(e6)*(cos(e5)*(cos(e1)*sin(e4) - sin(e2 + e3)*cos(e4)*sin(e1)) - cos(e2 + e3)*sin(e1)*sin(e5))) - y6*(cos(e6)*(cos(e1)*cos(e4) + sin(e2 + e3)*sin(e1)*sin(e4)) - sin(e6)*(cos(e5)*(cos(e1)*sin(e4) - sin(e2 + e3)*cos(e4)*sin(e1)) - cos(e2 + e3)*sin(e1)*sin(e5))) + z6*(sin(e5)*(cos(e1)*sin(e4) - sin(e2 + e3)*cos(e4)*sin(e1)) + cos(e2 + e3)*cos(e5)*sin(e1))),I6yz*cos(e4)*cos(e6) + I6zx*cos(e4)*sin(e6) + I6zz*sin(e4)*sin(e5) + I6zx*cos(e5)*cos(e6)*sin(e4) - I6yz*cos(e5)*sin(e4)*sin(e6) + m6*x6^2*sin(e4)*sin(e5) + m6*y6^2*sin(e4)*sin(e5) - a3*m6*y6*cos(e6)*sin(e5) + d4*m6*x6*cos(e6)*sin(e4) + m6*y6*z6*cos(e4)*cos(e6) - a3*m6*x6*sin(e5)*sin(e6) - d4*m6*y6*sin(e4)*sin(e6) + m6*x6*z6*cos(e4)*sin(e6) + d4*m6*y6*cos(e4)*cos(e5)*cos(e6) - a2*m6*y6*cos(e3)*cos(e6)*sin(e5) + d4*m6*x6*cos(e4)*cos(e5)*sin(e6) - a2*m6*x6*cos(e6)*sin(e3)*sin(e4) - a2*m6*x6*cos(e3)*sin(e5)*sin(e6) + m6*x6*z6*cos(e5)*cos(e6)*sin(e4) + a2*m6*y6*sin(e3)*sin(e4)*sin(e6) - m6*y6*z6*cos(e5)*sin(e4)*sin(e6) - a2*m6*y6*cos(e4)*cos(e5)*cos(e6)*sin(e3) - a2*m6*x6*cos(e4)*cos(e5)*sin(e3)*sin(e6),I6yz*cos(e4)*cos(e6) + I6zx*cos(e4)*sin(e6) + I6zz*sin(e4)*sin(e5) + I6zx*cos(e5)*cos(e6)*sin(e4) - I6yz*cos(e5)*sin(e4)*sin(e6) + m6*x6^2*sin(e4)*sin(e5) + m6*y6^2*sin(e4)*sin(e5) - a3*m6*y6*cos(e6)*sin(e5) + d4*m6*x6*cos(e6)*sin(e4) + m6*y6*z6*cos(e4)*cos(e6) - a3*m6*x6*sin(e5)*sin(e6) - d4*m6*y6*sin(e4)*sin(e6) + m6*x6*z6*cos(e4)*sin(e6) + d4*m6*y6*cos(e4)*cos(e5)*cos(e6) + d4*m6*x6*cos(e4)*cos(e5)*sin(e6) + m6*x6*z6*cos(e5)*cos(e6)*sin(e4) - m6*y6*z6*cos(e5)*sin(e4)*sin(e6),I6zz*cos(e5) - I6zx*cos(e6)*sin(e5) + I6yz*sin(e5)*sin(e6) + m6*x6^2*cos(e5) + m6*y6^2*cos(e5) - m6*x6*z6*cos(e6)*sin(e5) + m6*y6*z6*sin(e5)*sin(e6),I6yz*cos(e6) + I6zx*sin(e6) + m6*y6*z6*cos(e6) + m6*x6*z6*sin(e6),I6zz + m6*x6^2 + m6*y6^2];

C = ...
